simulink model "model"  (R2014a)
(part 3 of 3)

  powergui : powerlib/powergui  Priority=1  SimulationMode=Continuous  SolverType=Tustin  SampleTime=50e-6  frequency=60  SPID=off  DisableSnubberDevices=off  DisableRonSwitches=off  DisableVfSwitches=off  SwTol=0  Interpol=off  DisplayEquations=off  Ts=0  methode=off  frequencyindice=60  Pbase=100e6  ErrMax=1e-4  Iterations=50  UnitsV=kV  UnitsW=MW  FunctionMessages=off  echomessages=off  HookPort=off  EnableUseOfTLC=off  x0status=blocks  RestoreLinks=warning  ResistiveCurrentMeasurement=off  Frange=[0:2:500]  Ylog=off  Xlog=on  ShowGrid=off  save=off  variable=ZData  structure=0  ZoomFFT=off  StartTime=0.0  cycles=1  DisplayStyle=1  fundamental=60  FreqAxis=off  MaxFrequency=1000  frequencyindicesteady=1  RmsSteady=1  display=off
  ВЛ_110_кВ_ВТГРЭС___ПС_Рудянка_CN_276394749_110000_CN_188857424_110000 : powerlib/Elements/Distributed Parameters Line  Phases=3  Frequency=60  Resistance=[0.01273 0.3864]  Inductance="[0.9337e-3  4.1264e-3]"  Capacitance=[12.74e-9 7.751e-9]  Length=27.2985  x1=[0 0 0 0; 0.0001244 0 0 0; 0.0002488 0 0 0; 0.0003733 0 0 0; 0.0004977 0 0 0; 0.0006221 0 0 0]  x2=[0 0 0 0; 0.0001244 0 0 0; 0.0002488 0 0 0; 0.0003733 0 0 0; 0.0004977 0 0 0; 0.0006221 0 0 0]  x3=[0 0 0 0; 0.0001244 0 0 0; 0.0002488 0 0 0; 0.0003733 0 0 0; 0.0004977 0 0 0; 0.0006221 0 0 0]  x4=[0 0 0 0; 0.0001244 0 0 0; 0.0002488 0 0 0; 0.0003733 0 0 0; 0.0004977 0 0 0; 0.0006221 0 0 0]  x5=0  V1=ones(3,3)  V2=ones(3,3)  I1=ones(3,3)  I2=ones(3,3)  nHarmo=1  Measurements=None
  ВЛ_110_кВ_Верховино_Успенка_CN_174028758_110000_CN_277716444_110000 : powerlib/Elements/Distributed Parameters Line  Phases=3  Frequency=60  Resistance=[0.01273 0.3864]  Inductance="[0.9337e-3  4.1264e-3]"  Capacitance=[12.74e-9 7.751e-9]  Length=31.6484  x1=[0 0 0 0; 0.0001244 0 0 0; 0.0002488 0 0 0; 0.0003733 0 0 0; 0.0004977 0 0 0; 0.0006221 0 0 0]  x2=[0 0 0 0; 0.0001244 0 0 0; 0.0002488 0 0 0; 0.0003733 0 0 0; 0.0004977 0 0 0; 0.0006221 0 0 0]  x3=[0 0 0 0; 0.0001244 0 0 0; 0.0002488 0 0 0; 0.0003733 0 0 0; 0.0004977 0 0 0; 0.0006221 0 0 0]  x4=[0 0 0 0; 0.0001244 0 0 0; 0.0002488 0 0 0; 0.0003733 0 0 0; 0.0004977 0 0 0; 0.0006221 0 0 0]  x5=0  V1=ones(3,3)  V2=ones(3,3)  I1=ones(3,3)  I2=ones(3,3)  nHarmo=1  Measurements=None
  ВЛ_110_кВ_Новогеоргиевская___Княженская_CN_373906159_110000_CN_144699678_110000 : powerlib/Elements/Distributed Parameters Line  Phases=3  Frequency=60  Resistance=[0.01273 0.3864]  Inductance="[0.9337e-3  4.1264e-3]"  Capacitance=[12.74e-9 7.751e-9]  Length=16.9419  x1=[0 0 0 0; 0.0001244 0 0 0; 0.0002488 0 0 0; 0.0003733 0 0 0; 0.0004977 0 0 0; 0.0006221 0 0 0]  x2=[0 0 0 0; 0.0001244 0 0 0; 0.0002488 0 0 0; 0.0003733 0 0 0; 0.0004977 0 0 0; 0.0006221 0 0 0]  x3=[0 0 0 0; 0.0001244 0 0 0; 0.0002488 0 0 0; 0.0003733 0 0 0; 0.0004977 0 0 0; 0.0006221 0 0 0]  x4=[0 0 0 0; 0.0001244 0 0 0; 0.0002488 0 0 0; 0.0003733 0 0 0; 0.0004977 0 0 0; 0.0006221 0 0 0]  x5=0  V1=ones(3,3)  V2=ones(3,3)  I1=ones(3,3)  I2=ones(3,3)  nHarmo=1  Measurements=None
  ВЛ_110_кВ_Окунево___Солнечная_1_CN_273707087_110000_CN_110538007_110000 : powerlib/Elements/Distributed Parameters Line  Phases=3  Frequency=60  Resistance=[0.01273 0.3864]  Inductance="[0.9337e-3  4.1264e-3]"  Capacitance=[12.74e-9 7.751e-9]  Length=7.7084  x1=[0 0 0 0; 0.0001244 0 0 0; 0.0002488 0 0 0; 0.0003733 0 0 0; 0.0004977 0 0 0; 0.0006221 0 0 0]  x2=[0 0 0 0; 0.0001244 0 0 0; 0.0002488 0 0 0; 0.0003733 0 0 0; 0.0004977 0 0 0; 0.0006221 0 0 0]  x3=[0 0 0 0; 0.0001244 0 0 0; 0.0002488 0 0 0; 0.0003733 0 0 0; 0.0004977 0 0 0; 0.0006221 0 0 0]  x4=[0 0 0 0; 0.0001244 0 0 0; 0.0002488 0 0 0; 0.0003733 0 0 0; 0.0004977 0 0 0; 0.0006221 0 0 0]  x5=0  V1=ones(3,3)  V2=ones(3,3)  I1=ones(3,3)  I2=ones(3,3)  nHarmo=1  Measurements=None
  ВЛ_110_кВ_ПС_Зарница___ПС_Тугулым_CN_229397794_110000_CN_279664558_110000 : powerlib/Elements/Distributed Parameters Line  Phases=3  Frequency=60  Resistance=[0.01273 0.3864]  Inductance="[0.9337e-3  4.1264e-3]"  Capacitance=[12.74e-9 7.751e-9]  Length=22.5038  x1=[0 0 0 0; 0.0001244 0 0 0; 0.0002488 0 0 0; 0.0003733 0 0 0; 0.0004977 0 0 0; 0.0006221 0 0 0]  x2=[0 0 0 0; 0.0001244 0 0 0; 0.0002488 0 0 0; 0.0003733 0 0 0; 0.0004977 0 0 0; 0.0006221 0 0 0]  x3=[0 0 0 0; 0.0001244 0 0 0; 0.0002488 0 0 0; 0.0003733 0 0 0; 0.0004977 0 0 0; 0.0006221 0 0 0]  x4=[0 0 0 0; 0.0001244 0 0 0; 0.0002488 0 0 0; 0.0003733 0 0 0; 0.0004977 0 0 0; 0.0006221 0 0 0]  x5=0  V1=ones(3,3)  V2=ones(3,3)  I1=ones(3,3)  I2=ones(3,3)  nHarmo=1  Measurements=None
  ВЛ_110_кВ_ПС_Кармак___ПС_Верховино_CN_279664559_110000_CN_174028758_110000 : powerlib/Elements/Distributed Parameters Line  Phases=3  Frequency=60  Resistance=[0.01273 0.3864]  Inductance="[0.9337e-3  4.1264e-3]"  Capacitance=[12.74e-9 7.751e-9]  Length=5.7456  x1=[0 0 0 0; 0.0001244 0 0 0; 0.0002488 0 0 0; 0.0003733 0 0 0; 0.0004977 0 0 0; 0.0006221 0 0 0]  x2=[0 0 0 0; 0.0001244 0 0 0; 0.0002488 0 0 0; 0.0003733 0 0 0; 0.0004977 0 0 0; 0.0006221 0 0 0]  x3=[0 0 0 0; 0.0001244 0 0 0; 0.0002488 0 0 0; 0.0003733 0 0 0; 0.0004977 0 0 0; 0.0006221 0 0 0]  x4=[0 0 0 0; 0.0001244 0 0 0; 0.0002488 0 0 0; 0.0003733 0 0 0; 0.0004977 0 0 0; 0.0006221 0 0 0]  x5=0  V1=ones(3,3)  V2=ones(3,3)  I1=ones(3,3)  I2=ones(3,3)  nHarmo=1  Measurements=None
  ВЛ_110_кВ_ПС_Краснотурьинск___ПС_Североуральск_CN_281458614_110000_CN_281458615_110000 : powerlib/Elements/Distributed Parameters Line  Phases=3  Frequency=60  Resistance=[0.01273 0.3864]  Inductance="[0.9337e-3  4.1264e-3]"  Capacitance=[12.74e-9 7.751e-9]  Length=3.8522  x1=[0 0 0 0; 0.0001244 0 0 0; 0.0002488 0 0 0; 0.0003733 0 0 0; 0.0004977 0 0 0; 0.0006221 0 0 0]  x2=[0 0 0 0; 0.0001244 0 0 0; 0.0002488 0 0 0; 0.0003733 0 0 0; 0.0004977 0 0 0; 0.0006221 0 0 0]  x3=[0 0 0 0; 0.0001244 0 0 0; 0.0002488 0 0 0; 0.0003733 0 0 0; 0.0004977 0 0 0; 0.0006221 0 0 0]  x4=[0 0 0 0; 0.0001244 0 0 0; 0.0002488 0 0 0; 0.0003733 0 0 0; 0.0004977 0 0 0; 0.0006221 0 0 0]  x5=0  V1=ones(3,3)  V2=ones(3,3)  I1=ones(3,3)  I2=ones(3,3)  nHarmo=1  Measurements=None
  ВЛ_110_кВ_ПС_Черемухово___ПС_Першино_CN_235846243_110000_CN_281707739_110000 : powerlib/Elements/Distributed Parameters Line  Phases=3  Frequency=60  Resistance=[0.01273 0.3864]  Inductance="[0.9337e-3  4.1264e-3]"  Capacitance=[12.74e-9 7.751e-9]  Length=9.1519  x1=[0 0 0 0; 0.0001244 0 0 0; 0.0002488 0 0 0; 0.0003733 0 0 0; 0.0004977 0 0 0; 0.0006221 0 0 0]  x2=[0 0 0 0; 0.0001244 0 0 0; 0.0002488 0 0 0; 0.0003733 0 0 0; 0.0004977 0 0 0; 0.0006221 0 0 0]  x3=[0 0 0 0; 0.0001244 0 0 0; 0.0002488 0 0 0; 0.0003733 0 0 0; 0.0004977 0 0 0; 0.0006221 0 0 0]  x4=[0 0 0 0; 0.0001244 0 0 0; 0.0002488 0 0 0; 0.0003733 0 0 0; 0.0004977 0 0 0; 0.0006221 0 0 0]  x5=0  V1=ones(3,3)  V2=ones(3,3)  I1=ones(3,3)  I2=ones(3,3)  nHarmo=1  Measurements=None
  ВЛ_110_кВ_ПС_Черноисточинск___ПС_НЦЗ_CN_105584274_110000_CN_274851642_110000 : powerlib/Elements/Distributed Parameters Line  Phases=3  Frequency=60  Resistance=[0.01273 0.3864]  Inductance="[0.9337e-3  4.1264e-3]"  Capacitance=[12.74e-9 7.751e-9]  Length=49.7933  x1=[0 0 0 0; 0.0001244 0 0 0; 0.0002488 0 0 0; 0.0003733 0 0 0; 0.0004977 0 0 0; 0.0006221 0 0 0]  x2=[0 0 0 0; 0.0001244 0 0 0; 0.0002488 0 0 0; 0.0003733 0 0 0; 0.0004977 0 0 0; 0.0006221 0 0 0]  x3=[0 0 0 0; 0.0001244 0 0 0; 0.0002488 0 0 0; 0.0003733 0 0 0; 0.0004977 0 0 0; 0.0006221 0 0 0]  x4=[0 0 0 0; 0.0001244 0 0 0; 0.0002488 0 0 0; 0.0003733 0 0 0; 0.0004977 0 0 0; 0.0006221 0 0 0]  x5=0  V1=ones(3,3)  V2=ones(3,3)  I1=ones(3,3)  I2=ones(3,3)  nHarmo=1  Measurements=None
  ВЛ_110_кВ_ПС_Школьная___ПС_Рудянка_CN_275095838_110000_CN_276394749_110000 : powerlib/Elements/Distributed Parameters Line  Phases=3  Frequency=60  Resistance=[0.01273 0.3864]  Inductance="[0.9337e-3  4.1264e-3]"  Capacitance=[12.74e-9 7.751e-9]  Length=22.0688  x1=[0 0 0 0; 0.0001244 0 0 0; 0.0002488 0 0 0; 0.0003733 0 0 0; 0.0004977 0 0 0; 0.0006221 0 0 0]  x2=[0 0 0 0; 0.0001244 0 0 0; 0.0002488 0 0 0; 0.0003733 0 0 0; 0.0004977 0 0 0; 0.0006221 0 0 0]  x3=[0 0 0 0; 0.0001244 0 0 0; 0.0002488 0 0 0; 0.0003733 0 0 0; 0.0004977 0 0 0; 0.0006221 0 0 0]  x4=[0 0 0 0; 0.0001244 0 0 0; 0.0002488 0 0 0; 0.0003733 0 0 0; 0.0004977 0 0 0; 0.0006221 0 0 0]  x5=0  V1=ones(3,3)  V2=ones(3,3)  I1=ones(3,3)  I2=ones(3,3)  nHarmo=1  Measurements=None
  ВЛ_110_кВ_ПС_Юшала___ПС_Яр_CN_200241256_110000_CN_279664560_110000 : powerlib/Elements/Distributed Parameters Line  Phases=3  Frequency=60  Resistance=[0.01273 0.3864]  Inductance="[0.9337e-3  4.1264e-3]"  Capacitance=[12.74e-9 7.751e-9]  Length=16.032  x1=[0 0 0 0; 0.0001244 0 0 0; 0.0002488 0 0 0; 0.0003733 0 0 0; 0.0004977 0 0 0; 0.0006221 0 0 0]  x2=[0 0 0 0; 0.0001244 0 0 0; 0.0002488 0 0 0; 0.0003733 0 0 0; 0.0004977 0 0 0; 0.0006221 0 0 0]  x3=[0 0 0 0; 0.0001244 0 0 0; 0.0002488 0 0 0; 0.0003733 0 0 0; 0.0004977 0 0 0; 0.0006221 0 0 0]  x4=[0 0 0 0; 0.0001244 0 0 0; 0.0002488 0 0 0; 0.0003733 0 0 0; 0.0004977 0 0 0; 0.0006221 0 0 0]  x5=0  V1=ones(3,3)  V2=ones(3,3)  I1=ones(3,3)  I2=ones(3,3)  nHarmo=1  Measurements=None
  ВЛ_110_кВ_ПС_Яр___ПС_Истоур_CN_200241256_110000_CN_280145603_110000 : powerlib/Elements/Distributed Parameters Line  Phases=3  Frequency=60  Resistance=[0.01273 0.3864]  Inductance="[0.9337e-3  4.1264e-3]"  Capacitance=[12.74e-9 7.751e-9]  Length=35.0943  x1=[0 0 0 0; 0.0001244 0 0 0; 0.0002488 0 0 0; 0.0003733 0 0 0; 0.0004977 0 0 0; 0.0006221 0 0 0]  x2=[0 0 0 0; 0.0001244 0 0 0; 0.0002488 0 0 0; 0.0003733 0 0 0; 0.0004977 0 0 0; 0.0006221 0 0 0]  x3=[0 0 0 0; 0.0001244 0 0 0; 0.0002488 0 0 0; 0.0003733 0 0 0; 0.0004977 0 0 0; 0.0006221 0 0 0]  x4=[0 0 0 0; 0.0001244 0 0 0; 0.0002488 0 0 0; 0.0003733 0 0 0; 0.0004977 0 0 0; 0.0006221 0 0 0]  x5=0  V1=ones(3,3)  V2=ones(3,3)  I1=ones(3,3)  I2=ones(3,3)  nHarmo=1  Measurements=None
  ВЛ_110_кВ_СУГРЭС___ПС_Школьная_CN_275095838_110000_CN_131114928_110000 : powerlib/Elements/Distributed Parameters Line  Phases=3  Frequency=60  Resistance=[0.01273 0.3864]  Inductance="[0.9337e-3  4.1264e-3]"  Capacitance=[12.74e-9 7.751e-9]  Length=53.717  x1=[0 0 0 0; 0.0001244 0 0 0; 0.0002488 0 0 0; 0.0003733 0 0 0; 0.0004977 0 0 0; 0.0006221 0 0 0]  x2=[0 0 0 0; 0.0001244 0 0 0; 0.0002488 0 0 0; 0.0003733 0 0 0; 0.0004977 0 0 0; 0.0006221 0 0 0]  x3=[0 0 0 0; 0.0001244 0 0 0; 0.0002488 0 0 0; 0.0003733 0 0 0; 0.0004977 0 0 0; 0.0006221 0 0 0]  x4=[0 0 0 0; 0.0001244 0 0 0; 0.0002488 0 0 0; 0.0003733 0 0 0; 0.0004977 0 0 0; 0.0006221 0 0 0]  x5=0  V1=ones(3,3)  V2=ones(3,3)  I1=ones(3,3)  I2=ones(3,3)  nHarmo=1  Measurements=None
  ВЛ_110_кВ_СУГРЭС___ПС_Школьная_CN_275095838_110000_CN_317157140_110000 : powerlib/Elements/Distributed Parameters Line  Phases=3  Frequency=60  Resistance=[0.01273 0.3864]  Inductance="[0.9337e-3  4.1264e-3]"  Capacitance=[12.74e-9 7.751e-9]  Length=32.9199  x1=[0 0 0 0; 0.0001244 0 0 0; 0.0002488 0 0 0; 0.0003733 0 0 0; 0.0004977 0 0 0; 0.0006221 0 0 0]  x2=[0 0 0 0; 0.0001244 0 0 0; 0.0002488 0 0 0; 0.0003733 0 0 0; 0.0004977 0 0 0; 0.0006221 0 0 0]  x3=[0 0 0 0; 0.0001244 0 0 0; 0.0002488 0 0 0; 0.0003733 0 0 0; 0.0004977 0 0 0; 0.0006221 0 0 0]  x4=[0 0 0 0; 0.0001244 0 0 0; 0.0002488 0 0 0; 0.0003733 0 0 0; 0.0004977 0 0 0; 0.0006221 0 0 0]  x5=0  V1=ones(3,3)  V2=ones(3,3)  I1=ones(3,3)  I2=ones(3,3)  nHarmo=1  Measurements=None
  ВЛ_110_кВ_СУГРЭС___ПС_Школьная_CN_275095838_110000_CN_37479179_110000 : powerlib/Elements/Distributed Parameters Line  Phases=3  Frequency=60  Resistance=[0.01273 0.3864]  Inductance="[0.9337e-3  4.1264e-3]"  Capacitance=[12.74e-9 7.751e-9]  Length=30.521  x1=[0 0 0 0; 0.0001244 0 0 0; 0.0002488 0 0 0; 0.0003733 0 0 0; 0.0004977 0 0 0; 0.0006221 0 0 0]  x2=[0 0 0 0; 0.0001244 0 0 0; 0.0002488 0 0 0; 0.0003733 0 0 0; 0.0004977 0 0 0; 0.0006221 0 0 0]  x3=[0 0 0 0; 0.0001244 0 0 0; 0.0002488 0 0 0; 0.0003733 0 0 0; 0.0004977 0 0 0; 0.0006221 0 0 0]  x4=[0 0 0 0; 0.0001244 0 0 0; 0.0002488 0 0 0; 0.0003733 0 0 0; 0.0004977 0 0 0; 0.0006221 0 0 0]  x5=0  V1=ones(3,3)  V2=ones(3,3)  I1=ones(3,3)  I2=ones(3,3)  nHarmo=1  Measurements=None
  ВЛ_110_кВ_СУГРЭС___ПС_Школьная_CN_275095838_110000_CN_66264428_110000 : powerlib/Elements/Distributed Parameters Line  Phases=3  Frequency=60  Resistance=[0.01273 0.3864]  Inductance="[0.9337e-3  4.1264e-3]"  Capacitance=[12.74e-9 7.751e-9]  Length=36.1648  x1=[0 0 0 0; 0.0001244 0 0 0; 0.0002488 0 0 0; 0.0003733 0 0 0; 0.0004977 0 0 0; 0.0006221 0 0 0]  x2=[0 0 0 0; 0.0001244 0 0 0; 0.0002488 0 0 0; 0.0003733 0 0 0; 0.0004977 0 0 0; 0.0006221 0 0 0]  x3=[0 0 0 0; 0.0001244 0 0 0; 0.0002488 0 0 0; 0.0003733 0 0 0; 0.0004977 0 0 0; 0.0006221 0 0 0]  x4=[0 0 0 0; 0.0001244 0 0 0; 0.0002488 0 0 0; 0.0003733 0 0 0; 0.0004977 0 0 0; 0.0006221 0 0 0]  x5=0  V1=ones(3,3)  V2=ones(3,3)  I1=ones(3,3)  I2=ones(3,3)  nHarmo=1  Measurements=None
  ВЛ_110_кВ_СУГРЭС___ПС_Школьная_CN_275095838_110000_CN_76449471_110000 : powerlib/Elements/Distributed Parameters Line  Phases=3  Frequency=60  Resistance=[0.01273 0.3864]  Inductance="[0.9337e-3  4.1264e-3]"  Capacitance=[12.74e-9 7.751e-9]  Length=48.8137  x1=[0 0 0 0; 0.0001244 0 0 0; 0.0002488 0 0 0; 0.0003733 0 0 0; 0.0004977 0 0 0; 0.0006221 0 0 0]  x2=[0 0 0 0; 0.0001244 0 0 0; 0.0002488 0 0 0; 0.0003733 0 0 0; 0.0004977 0 0 0; 0.0006221 0 0 0]  x3=[0 0 0 0; 0.0001244 0 0 0; 0.0002488 0 0 0; 0.0003733 0 0 0; 0.0004977 0 0 0; 0.0006221 0 0 0]  x4=[0 0 0 0; 0.0001244 0 0 0; 0.0002488 0 0 0; 0.0003733 0 0 0; 0.0004977 0 0 0; 0.0006221 0 0 0]  x5=0  V1=ones(3,3)  V2=ones(3,3)  I1=ones(3,3)  I2=ones(3,3)  nHarmo=1  Measurements=None
  ВЛ_110кВ_Кр_Горка_Арси_CN_250194000_110000_CN_191446930_110000 : powerlib/Elements/Distributed Parameters Line  Phases=3  Frequency=60  Resistance=[0.01273 0.3864]  Inductance="[0.9337e-3  4.1264e-3]"  Capacitance=[12.74e-9 7.751e-9]  Length=30.043  x1=[0 0 0 0; 0.0001244 0 0 0; 0.0002488 0 0 0; 0.0003733 0 0 0; 0.0004977 0 0 0; 0.0006221 0 0 0]  x2=[0 0 0 0; 0.0001244 0 0 0; 0.0002488 0 0 0; 0.0003733 0 0 0; 0.0004977 0 0 0; 0.0006221 0 0 0]  x3=[0 0 0 0; 0.0001244 0 0 0; 0.0002488 0 0 0; 0.0003733 0 0 0; 0.0004977 0 0 0; 0.0006221 0 0 0]  x4=[0 0 0 0; 0.0001244 0 0 0; 0.0002488 0 0 0; 0.0003733 0 0 0; 0.0004977 0 0 0; 0.0006221 0 0 0]  x5=0  V1=ones(3,3)  V2=ones(3,3)  I1=ones(3,3)  I2=ones(3,3)  nHarmo=1  Measurements=None
  ВЛ_110кВ_Кр_Горка_Березинская_CN_314008364_110000_CN_191446930_110000 : powerlib/Elements/Distributed Parameters Line  Phases=3  Frequency=60  Resistance=[0.01273 0.3864]  Inductance="[0.9337e-3  4.1264e-3]"  Capacitance=[12.74e-9 7.751e-9]  Length=23.6796  x1=[0 0 0 0; 0.0001244 0 0 0; 0.0002488 0 0 0; 0.0003733 0 0 0; 0.0004977 0 0 0; 0.0006221 0 0 0]  x2=[0 0 0 0; 0.0001244 0 0 0; 0.0002488 0 0 0; 0.0003733 0 0 0; 0.0004977 0 0 0; 0.0006221 0 0 0]  x3=[0 0 0 0; 0.0001244 0 0 0; 0.0002488 0 0 0; 0.0003733 0 0 0; 0.0004977 0 0 0; 0.0006221 0 0 0]  x4=[0 0 0 0; 0.0001244 0 0 0; 0.0002488 0 0 0; 0.0003733 0 0 0; 0.0004977 0 0 0; 0.0006221 0 0 0]  x5=0  V1=ones(3,3)  V2=ones(3,3)  I1=ones(3,3)  I2=ones(3,3)  nHarmo=1  Measurements=None
  ВЛ_110кВ_ПС90_Кр_Горка_отпайка_на_Фершампенуаз_CN_199389117_110000_CN_191446930_110000 : powerlib/Elements/Distributed Parameters Line  Phases=3  Frequency=60  Resistance=[0.01273 0.3864]  Inductance="[0.9337e-3  4.1264e-3]"  Capacitance=[12.74e-9 7.751e-9]  Length=19.2536  x1=[0 0 0 0; 0.0001244 0 0 0; 0.0002488 0 0 0; 0.0003733 0 0 0; 0.0004977 0 0 0; 0.0006221 0 0 0]  x2=[0 0 0 0; 0.0001244 0 0 0; 0.0002488 0 0 0; 0.0003733 0 0 0; 0.0004977 0 0 0; 0.0006221 0 0 0]  x3=[0 0 0 0; 0.0001244 0 0 0; 0.0002488 0 0 0; 0.0003733 0 0 0; 0.0004977 0 0 0; 0.0006221 0 0 0]  x4=[0 0 0 0; 0.0001244 0 0 0; 0.0002488 0 0 0; 0.0003733 0 0 0; 0.0004977 0 0 0; 0.0006221 0 0 0]  x5=0  V1=ones(3,3)  V2=ones(3,3)  I1=ones(3,3)  I2=ones(3,3)  nHarmo=1  Measurements=None
  ВЛ_110кВ_ПС90_Кр_Горка_отпайка_на_Фершампенуаз_CN_199389117_110000_CN_339193644_110000 : powerlib/Elements/Distributed Parameters Line  Phases=3  Frequency=60  Resistance=[0.01273 0.3864]  Inductance="[0.9337e-3  4.1264e-3]"  Capacitance=[12.74e-9 7.751e-9]  Length=37.4111  x1=[0 0 0 0; 0.0001244 0 0 0; 0.0002488 0 0 0; 0.0003733 0 0 0; 0.0004977 0 0 0; 0.0006221 0 0 0]  x2=[0 0 0 0; 0.0001244 0 0 0; 0.0002488 0 0 0; 0.0003733 0 0 0; 0.0004977 0 0 0; 0.0006221 0 0 0]  x3=[0 0 0 0; 0.0001244 0 0 0; 0.0002488 0 0 0; 0.0003733 0 0 0; 0.0004977 0 0 0; 0.0006221 0 0 0]  x4=[0 0 0 0; 0.0001244 0 0 0; 0.0002488 0 0 0; 0.0003733 0 0 0; 0.0004977 0 0 0; 0.0006221 0 0 0]  x5=0  V1=ones(3,3)  V2=ones(3,3)  I1=ones(3,3)  I2=ones(3,3)  nHarmo=1  Measurements=None
  ВЛ_220_кВ_ПС_БАЗ___ПС_Белка_CN_300566433_220000_CN_108718929_220000 : powerlib/Elements/Distributed Parameters Line  Phases=3  Frequency=60  Resistance=[0.01273 0.3864]  Inductance="[0.9337e-3  4.1264e-3]"  Capacitance=[12.74e-9 7.751e-9]  Length=8.0242  x1=[0 0 0 0; 0.0001244 0 0 0; 0.0002488 0 0 0; 0.0003733 0 0 0; 0.0004977 0 0 0; 0.0006221 0 0 0]  x2=[0 0 0 0; 0.0001244 0 0 0; 0.0002488 0 0 0; 0.0003733 0 0 0; 0.0004977 0 0 0; 0.0006221 0 0 0]  x3=[0 0 0 0; 0.0001244 0 0 0; 0.0002488 0 0 0; 0.0003733 0 0 0; 0.0004977 0 0 0; 0.0006221 0 0 0]  x4=[0 0 0 0; 0.0001244 0 0 0; 0.0002488 0 0 0; 0.0003733 0 0 0; 0.0004977 0 0 0; 0.0006221 0 0 0]  x5=0  V1=ones(3,3)  V2=ones(3,3)  I1=ones(3,3)  I2=ones(3,3)  nHarmo=1  Measurements=None
  ВЛ_220_кВ_Первомайская_–_Салда_CN_274851651_220000_CN_107585072_220000 : powerlib/Elements/Distributed Parameters Line  Phases=3  Frequency=60  Resistance=[0.01273 0.3864]  Inductance="[0.9337e-3  4.1264e-3]"  Capacitance=[12.74e-9 7.751e-9]  Length=62.8508  x1=[0 0 0 0; 0.0001244 0 0 0; 0.0002488 0 0 0; 0.0003733 0 0 0; 0.0004977 0 0 0; 0.0006221 0 0 0]  x2=[0 0 0 0; 0.0001244 0 0 0; 0.0002488 0 0 0; 0.0003733 0 0 0; 0.0004977 0 0 0; 0.0006221 0 0 0]  x3=[0 0 0 0; 0.0001244 0 0 0; 0.0002488 0 0 0; 0.0003733 0 0 0; 0.0004977 0 0 0; 0.0006221 0 0 0]  x4=[0 0 0 0; 0.0001244 0 0 0; 0.0002488 0 0 0; 0.0003733 0 0 0; 0.0004977 0 0 0; 0.0006221 0 0 0]  x5=0  V1=ones(3,3)  V2=ones(3,3)  I1=ones(3,3)  I2=ones(3,3)  nHarmo=1  Measurements=None
  ВЛ_220_кВ_Троицкая_ГРЭС___Карталы_CN_96842811_220000_CN_109226934_220000 : powerlib/Elements/Distributed Parameters Line  Phases=3  Frequency=60  Resistance=[0.01273 0.3864]  Inductance="[0.9337e-3  4.1264e-3]"  Capacitance=[12.74e-9 7.751e-9]  Length=59.0733  x1=[0 0 0 0; 0.0001244 0 0 0; 0.0002488 0 0 0; 0.0003733 0 0 0; 0.0004977 0 0 0; 0.0006221 0 0 0]  x2=[0 0 0 0; 0.0001244 0 0 0; 0.0002488 0 0 0; 0.0003733 0 0 0; 0.0004977 0 0 0; 0.0006221 0 0 0]  x3=[0 0 0 0; 0.0001244 0 0 0; 0.0002488 0 0 0; 0.0003733 0 0 0; 0.0004977 0 0 0; 0.0006221 0 0 0]  x4=[0 0 0 0; 0.0001244 0 0 0; 0.0002488 0 0 0; 0.0003733 0 0 0; 0.0004977 0 0 0; 0.0006221 0 0 0]  x5=0  V1=ones(3,3)  V2=ones(3,3)  I1=ones(3,3)  I2=ones(3,3)  nHarmo=1  Measurements=None
  ВЛ_220кВ_Тр_ГРЭС_ПС90_1Л_CN_219112642_220000_CN_109226934_220000 : powerlib/Elements/Distributed Parameters Line  Phases=3  Frequency=60  Resistance=[0.01273 0.3864]  Inductance="[0.9337e-3  4.1264e-3]"  Capacitance=[12.74e-9 7.751e-9]  Length=57.6287  x1=[0 0 0 0; 0.0001244 0 0 0; 0.0002488 0 0 0; 0.0003733 0 0 0; 0.0004977 0 0 0; 0.0006221 0 0 0]  x2=[0 0 0 0; 0.0001244 0 0 0; 0.0002488 0 0 0; 0.0003733 0 0 0; 0.0004977 0 0 0; 0.0006221 0 0 0]  x3=[0 0 0 0; 0.0001244 0 0 0; 0.0002488 0 0 0; 0.0003733 0 0 0; 0.0004977 0 0 0; 0.0006221 0 0 0]  x4=[0 0 0 0; 0.0001244 0 0 0; 0.0002488 0 0 0; 0.0003733 0 0 0; 0.0004977 0 0 0; 0.0006221 0 0 0]  x5=0  V1=ones(3,3)  V2=ones(3,3)  I1=ones(3,3)  I2=ones(3,3)  nHarmo=1  Measurements=None
  ВЛ_500кВ_Кропачево___Приваловская_CN_169556579_500000_CN_113767652_500000 : powerlib/Elements/Distributed Parameters Line  Phases=3  Frequency=60  Resistance=[0.01273 0.3864]  Inductance="[0.9337e-3  4.1264e-3]"  Capacitance=[12.74e-9 7.751e-9]  Length=57.2159  x1=[0 0 0 0; 0.0001244 0 0 0; 0.0002488 0 0 0; 0.0003733 0 0 0; 0.0004977 0 0 0; 0.0006221 0 0 0]  x2=[0 0 0 0; 0.0001244 0 0 0; 0.0002488 0 0 0; 0.0003733 0 0 0; 0.0004977 0 0 0; 0.0006221 0 0 0]  x3=[0 0 0 0; 0.0001244 0 0 0; 0.0002488 0 0 0; 0.0003733 0 0 0; 0.0004977 0 0 0; 0.0006221 0 0 0]  x4=[0 0 0 0; 0.0001244 0 0 0; 0.0002488 0 0 0; 0.0003733 0 0 0; 0.0004977 0 0 0; 0.0006221 0 0 0]  x5=0  V1=ones(3,3)  V2=ones(3,3)  I1=ones(3,3)  I2=ones(3,3)  nHarmo=1  Measurements=None
  Отпайка_ВЛ_110_кВ_на_ПС_Твёрдые_сплавы_от_ВТГРЭС___Карпушиха_CN_276394758_110000_CN_188857424_110000 : powerlib/Elements/Distributed Parameters Line  Phases=3  Frequency=60  Resistance=[0.01273 0.3864]  Inductance="[0.9337e-3  4.1264e-3]"  Capacitance=[12.74e-9 7.751e-9]  Length=30.2501  x1=[0 0 0 0; 0.0001244 0 0 0; 0.0002488 0 0 0; 0.0003733 0 0 0; 0.0004977 0 0 0; 0.0006221 0 0 0]  x2=[0 0 0 0; 0.0001244 0 0 0; 0.0002488 0 0 0; 0.0003733 0 0 0; 0.0004977 0 0 0; 0.0006221 0 0 0]  x3=[0 0 0 0; 0.0001244 0 0 0; 0.0002488 0 0 0; 0.0003733 0 0 0; 0.0004977 0 0 0; 0.0006221 0 0 0]  x4=[0 0 0 0; 0.0001244 0 0 0; 0.0002488 0 0 0; 0.0003733 0 0 0; 0.0004977 0 0 0; 0.0006221 0 0 0]  x5=0  V1=ones(3,3)  V2=ones(3,3)  I1=ones(3,3)  I2=ones(3,3)  nHarmo=1  Measurements=None
  ПС_Таволги___ПС_Киприно___ПС_Черемисска_CN_273461546_110000_CN_101532642_110000 : powerlib/Elements/Distributed Parameters Line  Phases=3  Frequency=60  Resistance=[0.01273 0.3864]  Inductance="[0.9337e-3  4.1264e-3]"  Capacitance=[12.74e-9 7.751e-9]  Length=22.6465  x1=[0 0 0 0; 0.0001244 0 0 0; 0.0002488 0 0 0; 0.0003733 0 0 0; 0.0004977 0 0 0; 0.0006221 0 0 0]  x2=[0 0 0 0; 0.0001244 0 0 0; 0.0002488 0 0 0; 0.0003733 0 0 0; 0.0004977 0 0 0; 0.0006221 0 0 0]  x3=[0 0 0 0; 0.0001244 0 0 0; 0.0002488 0 0 0; 0.0003733 0 0 0; 0.0004977 0 0 0; 0.0006221 0 0 0]  x4=[0 0 0 0; 0.0001244 0 0 0; 0.0002488 0 0 0; 0.0003733 0 0 0; 0.0004977 0 0 0; 0.0006221 0 0 0]  x5=0  V1=ones(3,3)  V2=ones(3,3)  I1=ones(3,3)  I2=ones(3,3)  nHarmo=1  Measurements=None
  ПС_Таволги___ПС_Киприно___ПС_Черемисска_CN_273461546_110000_CN_135780398_110000 : powerlib/Elements/Distributed Parameters Line  Phases=3  Frequency=60  Resistance=[0.01273 0.3864]  Inductance="[0.9337e-3  4.1264e-3]"  Capacitance=[12.74e-9 7.751e-9]  Length=26.7512  x1=[0 0 0 0; 0.0001244 0 0 0; 0.0002488 0 0 0; 0.0003733 0 0 0; 0.0004977 0 0 0; 0.0006221 0 0 0]  x2=[0 0 0 0; 0.0001244 0 0 0; 0.0002488 0 0 0; 0.0003733 0 0 0; 0.0004977 0 0 0; 0.0006221 0 0 0]  x3=[0 0 0 0; 0.0001244 0 0 0; 0.0002488 0 0 0; 0.0003733 0 0 0; 0.0004977 0 0 0; 0.0006221 0 0 0]  x4=[0 0 0 0; 0.0001244 0 0 0; 0.0002488 0 0 0; 0.0003733 0 0 0; 0.0004977 0 0 0; 0.0006221 0 0 0]  x5=0  V1=ones(3,3)  V2=ones(3,3)  I1=ones(3,3)  I2=ones(3,3)  nHarmo=1  Measurements=None
  ПС_Таволги___ПС_Киприно___ПС_Черемисска_CN_273461546_110000_CN_273649961_110000 : powerlib/Elements/Distributed Parameters Line  Phases=3  Frequency=60  Resistance=[0.01273 0.3864]  Inductance="[0.9337e-3  4.1264e-3]"  Capacitance=[12.74e-9 7.751e-9]  Length=19.5309  x1=[0 0 0 0; 0.0001244 0 0 0; 0.0002488 0 0 0; 0.0003733 0 0 0; 0.0004977 0 0 0; 0.0006221 0 0 0]  x2=[0 0 0 0; 0.0001244 0 0 0; 0.0002488 0 0 0; 0.0003733 0 0 0; 0.0004977 0 0 0; 0.0006221 0 0 0]  x3=[0 0 0 0; 0.0001244 0 0 0; 0.0002488 0 0 0; 0.0003733 0 0 0; 0.0004977 0 0 0; 0.0006221 0 0 0]  x4=[0 0 0 0; 0.0001244 0 0 0; 0.0002488 0 0 0; 0.0003733 0 0 0; 0.0004977 0 0 0; 0.0006221 0 0 0]  x5=0  V1=ones(3,3)  V2=ones(3,3)  I1=ones(3,3)  I2=ones(3,3)  nHarmo=1  Measurements=None
  Тр_ГРЭС_Магнитогорск_CN_219112646_500000_CN_109226934_220000 : powerlib/Elements/Distributed Parameters Line  Phases=3  Frequency=60  Resistance=[0.01273 0.3864]  Inductance="[0.9337e-3  4.1264e-3]"  Capacitance=[12.74e-9 7.751e-9]  Length=9.2123  x1=[0 0 0 0; 0.0001244 0 0 0; 0.0002488 0 0 0; 0.0003733 0 0 0; 0.0004977 0 0 0; 0.0006221 0 0 0]  x2=[0 0 0 0; 0.0001244 0 0 0; 0.0002488 0 0 0; 0.0003733 0 0 0; 0.0004977 0 0 0; 0.0006221 0 0 0]  x3=[0 0 0 0; 0.0001244 0 0 0; 0.0002488 0 0 0; 0.0003733 0 0 0; 0.0004977 0 0 0; 0.0006221 0 0 0]  x4=[0 0 0 0; 0.0001244 0 0 0; 0.0002488 0 0 0; 0.0003733 0 0 0; 0.0004977 0 0 0; 0.0006221 0 0 0]  x5=0  V1=ones(3,3)  V2=ones(3,3)  I1=ones(3,3)  I2=ones(3,3)  nHarmo=1  Measurements=None
  connections:
  _CN_218733056_110000_CN_218733818_110000/LConn1 -- T_218733056__/LConn1 -- _CN_218733056_110000_CN_218733820_110000/LConn1
  _CN_218733056_110000_CN_218733818_110000/LConn2 -- T_218733056__/LConn2 -- _CN_218733056_110000_CN_218733820_110000/LConn2
  _CN_218733056_110000_CN_218733818_110000/LConn3 -- T_218733056__/LConn3 -- _CN_218733056_110000_CN_218733820_110000/LConn3 -- bus1/LConn1
  T_218733818__/LConn1 -- _CN_218733056_110000_CN_218733818_110000/RConn1
  T_218733818__/LConn2 -- _CN_218733056_110000_CN_218733818_110000/RConn2
  _CN_218733056_110000_CN_218733818_110000/RConn3 -- T_218733818__/LConn3 -- bus2/LConn1
  T_218733820__/LConn1 -- _CN_218733056_110000_CN_218733820_110000/RConn1
  T_218733820__/LConn2 -- _CN_218733056_110000_CN_218733820_110000/RConn2
  _CN_218733056_110000_CN_218733820_110000/RConn3 -- T_218733820__/LConn3 -- bus3/LConn1
  _CN_128448427_110000_CN_40080294_110000/LConn1 -- T_128448427__/LConn1 -- _CN_128448427_110000_CN_42918338_110000/LConn1 -- _CN_128448427_110000_CN_310639917_110000/LConn1 -- _CN_128448427_110000_CN_78488044_110000/LConn1 -- _CN_128448427_110000_CN_97827873_110000/LConn1
  _CN_128448427_110000_CN_40080294_110000/LConn2 -- T_128448427__/LConn2 -- _CN_128448427_110000_CN_42918338_110000/LConn2 -- _CN_128448427_110000_CN_310639917_110000/LConn2 -- _CN_128448427_110000_CN_78488044_110000/LConn2 -- _CN_128448427_110000_CN_97827873_110000/LConn2
  _CN_128448427_110000_CN_40080294_110000/LConn3 -- T_128448427__/LConn3 -- _CN_128448427_110000_CN_42918338_110000/LConn3 -- bus4/LConn1 -- _CN_128448427_110000_CN_310639917_110000/LConn3 -- _CN_128448427_110000_CN_78488044_110000/LConn3 -- _CN_128448427_110000_CN_97827873_110000/LConn3
  T_40080294_110000;10000_Московская/LConn1 -- _CN_128448427_110000_CN_40080294_110000/RConn1
  T_40080294_110000;10000_Московская/LConn2 -- _CN_128448427_110000_CN_40080294_110000/RConn2
  _CN_128448427_110000_CN_40080294_110000/RConn3 -- T_40080294_110000;10000_Московская/LConn3 -- bus5/LConn1
  T_310639917_110000;10000_Отрадная/LConn1 -- _CN_128448427_110000_CN_310639917_110000/RConn1
  T_310639917_110000;10000_Отрадная/LConn2 -- _CN_128448427_110000_CN_310639917_110000/RConn2
  _CN_128448427_110000_CN_310639917_110000/RConn3 -- T_310639917_110000;10000_Отрадная/LConn3 -- bus6/LConn1
  T_78488044__Академическая/LConn1 -- _CN_128448427_110000_CN_78488044_110000/RConn1
  T_78488044__Академическая/LConn2 -- _CN_128448427_110000_CN_78488044_110000/RConn2
  _CN_128448427_110000_CN_78488044_110000/RConn3 -- T_78488044__Академическая/LConn3 -- bus7/LConn1
  T_97827873__Овощная/LConn1 -- _CN_128448427_110000_CN_97827873_110000/RConn1
  T_97827873__Овощная/LConn2 -- _CN_128448427_110000_CN_97827873_110000/RConn2
  _CN_128448427_110000_CN_97827873_110000/RConn3 -- T_97827873__Овощная/LConn3 -- bus8/LConn1
  T_42918338__Ясная/LConn1 -- _CN_128448427_110000_CN_42918338_110000/RConn1
  T_42918338__Ясная/LConn2 -- _CN_128448427_110000_CN_42918338_110000/RConn2
  _CN_128448427_110000_CN_42918338_110000/RConn3 -- T_42918338__Ясная/LConn3 -- bus9/LConn1
  _CN_331102892_110000_CN_128346488_110000/LConn1 -- T_331102892__Бараба/LConn1 -- _CN_331102892_110000_CN_164371995_110000/LConn1 -- _CN_331102892_110000_CN_187971431_110000/LConn1 -- _CN_331102892_110000_CN_93050981_110000/LConn1
  _CN_331102892_110000_CN_128346488_110000/LConn2 -- T_331102892__Бараба/LConn2 -- _CN_331102892_110000_CN_164371995_110000/LConn2 -- _CN_331102892_110000_CN_187971431_110000/LConn2 -- _CN_331102892_110000_CN_93050981_110000/LConn2
  _CN_331102892_110000_CN_128346488_110000/LConn3 -- T_331102892__Бараба/LConn3 -- _CN_331102892_110000_CN_164371995_110000/LConn3 -- _CN_331102892_110000_CN_187971431_110000/LConn3 -- _CN_331102892_110000_CN_93050981_110000/LConn3 -- bus10/LConn1
  T_128346488__Грязновская/LConn1 -- _CN_331102892_110000_CN_128346488_110000/RConn1
  T_128346488__Грязновская/LConn2 -- _CN_331102892_110000_CN_128346488_110000/RConn2
  _CN_331102892_110000_CN_128346488_110000/RConn3 -- T_128346488__Грязновская/LConn3 -- bus11/LConn1
  T_164371995__/LConn1 -- _CN_331102892_110000_CN_164371995_110000/RConn1
  T_164371995__/LConn2 -- _CN_331102892_110000_CN_164371995_110000/RConn2
  _CN_331102892_110000_CN_164371995_110000/RConn3 -- T_164371995__/LConn3 -- bus12/LConn1
  T_187971431__Клевакино/LConn1 -- _CN_331102892_110000_CN_187971431_110000/RConn1
  T_187971431__Клевакино/LConn2 -- _CN_331102892_110000_CN_187971431_110000/RConn2
  _CN_331102892_110000_CN_187971431_110000/RConn3 -- T_187971431__Клевакино/LConn3 -- bus13/LConn1
  _CN_331102892_110000_CN_93050981_110000/RConn1 -- T_93050981__Черемхово/LConn1 -- _CN_320347053_110000_CN_93050981_110000/LConn1
  _CN_331102892_110000_CN_93050981_110000/RConn2 -- T_93050981__Черемхово/LConn2 -- _CN_320347053_110000_CN_93050981_110000/LConn2
  _CN_331102892_110000_CN_93050981_110000/RConn3 -- T_93050981__Черемхово/LConn3 -- _CN_320347053_110000_CN_93050981_110000/LConn3 -- bus14/LConn1
  T_320347053__Кочневское/LConn1 -- _CN_320347053_110000_CN_93050981_110000/RConn1
  T_320347053__Кочневское/LConn2 -- _CN_320347053_110000_CN_93050981_110000/RConn2
  _CN_320347053_110000_CN_93050981_110000/RConn3 -- T_320347053__Кочневское/LConn3 -- bus15/LConn1
  T_279497233__/LConn1 -- _CN_279497233_110000_CN_126093674_110000/LConn1
  T_279497233__/LConn2 -- _CN_279497233_110000_CN_126093674_110000/LConn2
  _CN_279497233_110000_CN_126093674_110000/LConn3 -- T_279497233__/LConn3 -- bus16/LConn1
  T_126093674__/LConn1 -- _CN_279497233_110000_CN_126093674_110000/RConn1
  T_126093674__/LConn2 -- _CN_279497233_110000_CN_126093674_110000/RConn2
  _CN_279497233_110000_CN_126093674_110000/RConn3 -- T_126093674__/LConn3 -- bus17/LConn1
  "T_96989715_110000;6000_ПС_\"Кварц\""/LConn1 -- _CN_96989715_110000_CN_93260139_110000/LConn1
  "T_96989715_110000;6000_ПС_\"Кварц\""/LConn2 -- _CN_96989715_110000_CN_93260139_110000/LConn2
  _CN_96989715_110000_CN_93260139_110000/LConn3 -- "T_96989715_110000;6000_ПС_\"Кварц\""/LConn3 -- bus18/LConn1
  T_93260139__Родник/LConn1 -- _CN_96989715_110000_CN_93260139_110000/RConn1
  T_93260139__Родник/LConn2 -- _CN_96989715_110000_CN_93260139_110000/RConn2
  _CN_96989715_110000_CN_93260139_110000/RConn3 -- T_93260139__Родник/LConn3 -- bus19/LConn1
  _CN_274652249_110000_CN_216208030_110000/LConn1 -- "T_274652249__П_ст_110_35_6кВ_\"Атиг\""/LConn1 -- _CN_274652249_110000_CN_106927870_110000/LConn1 -- _CN_274652249_110000_CN_255624915_110000/LConn1
  _CN_274652249_110000_CN_216208030_110000/LConn2 -- "T_274652249__П_ст_110_35_6кВ_\"Атиг\""/LConn2 -- _CN_274652249_110000_CN_106927870_110000/LConn2 -- _CN_274652249_110000_CN_255624915_110000/LConn2
  _CN_274652249_110000_CN_216208030_110000/LConn3 -- "T_274652249__П_ст_110_35_6кВ_\"Атиг\""/LConn3 -- _CN_274652249_110000_CN_106927870_110000/LConn3 -- _CN_274652249_110000_CN_255624915_110000/LConn3 -- bus20/LConn1
  "T_216208030_110000;35000;6000_ПС_\"Бисерть\""/LConn1 -- _CN_274652249_110000_CN_216208030_110000/RConn1
  "T_216208030_110000;35000;6000_ПС_\"Бисерть\""/LConn2 -- _CN_274652249_110000_CN_216208030_110000/RConn2
  _CN_274652249_110000_CN_216208030_110000/RConn3 -- "T_216208030_110000;35000;6000_ПС_\"Бисерть\""/LConn3 -- bus21/LConn1
  _CN_274652249_110000_CN_106927870_110000/RConn1 -- T_106927870__/LConn1 -- _CN_255624915_110000_CN_106927870_110000/LConn1
  _CN_274652249_110000_CN_106927870_110000/RConn2 -- T_106927870__/LConn2 -- _CN_255624915_110000_CN_106927870_110000/LConn2
  _CN_274652249_110000_CN_106927870_110000/RConn3 -- T_106927870__/LConn3 -- _CN_255624915_110000_CN_106927870_110000/LConn3 -- bus22/LConn1
  _CN_274652249_110000_CN_255624915_110000/RConn1 -- T_255624915__/LConn1 -- _CN_255624915_110000_CN_106927870_110000/RConn1
  _CN_274652249_110000_CN_255624915_110000/RConn2 -- T_255624915__/LConn2 -- _CN_255624915_110000_CN_106927870_110000/RConn2
  _CN_274652249_110000_CN_255624915_110000/RConn3 -- T_255624915__/LConn3 -- _CN_255624915_110000_CN_106927870_110000/RConn3 -- bus23/LConn1
  T_153740317_110000_ГОРНЫЙ_ЩИТ/LConn1 -- _CN_153740317_110000_CN_153741014_110000/LConn1
  T_153740317_110000_ГОРНЫЙ_ЩИТ/LConn2 -- _CN_153740317_110000_CN_153741014_110000/LConn2
  _CN_153740317_110000_CN_153741014_110000/LConn3 -- T_153740317_110000_ГОРНЫЙ_ЩИТ/LConn3 -- bus24/LConn1
  T_153741014__/LConn1 -- _CN_153740317_110000_CN_153741014_110000/RConn1
  T_153741014__/LConn2 -- _CN_153740317_110000_CN_153741014_110000/RConn2
  _CN_153740317_110000_CN_153741014_110000/RConn3 -- T_153741014__/LConn3 -- bus25/LConn1
  _CN_282779585_110000_CN_93418566_110000/LConn1 -- T_282779585__/LConn1 -- _CN_282779585_110000_CN_282779587_110000/LConn1
  _CN_282779585_110000_CN_93418566_110000/LConn2 -- T_282779585__/LConn2 -- _CN_282779585_110000_CN_282779587_110000/LConn2
  _CN_282779585_110000_CN_93418566_110000/LConn3 -- T_282779585__/LConn3 -- _CN_282779585_110000_CN_282779587_110000/LConn3 -- bus26/LConn1
  _CN_282779585_110000_CN_93418566_110000/RConn1 -- T_93418566_220000;110000_Травянская/RConn1 -- _CN_93418566_110000_CN_166188874_110000/LConn1 -- L_93418566/LConn1
  _CN_282779585_110000_CN_93418566_110000/RConn2 -- T_93418566_220000;110000_Травянская/RConn2 -- _CN_93418566_110000_CN_166188874_110000/LConn2 -- L_93418566/LConn2
  _CN_282779585_110000_CN_93418566_110000/RConn3 -- T_93418566_220000;110000_Травянская/RConn3 -- _CN_93418566_110000_CN_166188874_110000/LConn3 -- L_93418566/LConn3 -- bus27/LConn1
  T_282779587__/LConn1 -- _CN_282779585_110000_CN_282779587_110000/RConn1
  T_282779587__/LConn2 -- _CN_282779585_110000_CN_282779587_110000/RConn2
  _CN_282779585_110000_CN_282779587_110000/RConn3 -- T_282779587__/LConn3 -- bus28/LConn1
  T_282645278__/LConn1 -- _CN_282645278_110000_CN_166188874_110000/LConn1
  T_282645278__/LConn2 -- _CN_282645278_110000_CN_166188874_110000/LConn2
  _CN_282645278_110000_CN_166188874_110000/LConn3 -- T_282645278__/LConn3 -- bus29/LConn1
  _CN_282645278_110000_CN_166188874_110000/RConn1 -- T_166188874_220000;110000;10000_Каменская/RConn1 -- _CN_166188874_110000_CN_92045303_110000/LConn1 -- L_166188874/LConn1 -- _CN_166188874_110000_CN_282850239_110000/LConn1 -- _CN_166188874_110000_CN_282748778_110000/LConn1 -- _CN_93418566_110000_CN_166188874_110000/RConn1 -- _CN_280421437_110000_CN_166188874_110000/LConn1
  _CN_282645278_110000_CN_166188874_110000/RConn2 -- T_166188874_220000;110000;10000_Каменская/RConn2 -- _CN_166188874_110000_CN_92045303_110000/LConn2 -- L_166188874/LConn2 -- _CN_166188874_110000_CN_282850239_110000/LConn2 -- _CN_166188874_110000_CN_282748778_110000/LConn2 -- _CN_93418566_110000_CN_166188874_110000/RConn2 -- _CN_280421437_110000_CN_166188874_110000/LConn2
  _CN_282645278_110000_CN_166188874_110000/RConn3 -- T_166188874_220000;110000;10000_Каменская/RConn3 -- _CN_166188874_110000_CN_92045303_110000/LConn3 -- L_166188874/LConn3 -- bus30/LConn1 -- _CN_166188874_110000_CN_282850239_110000/LConn3 -- _CN_166188874_110000_CN_282748778_110000/LConn3 -- _CN_93418566_110000_CN_166188874_110000/RConn3 -- _CN_280421437_110000_CN_166188874_110000/LConn3
  _CN_121211432_110000_CN_372580506_110000/LConn1 -- T_121211432__Ильменская/LConn1 -- _CN_121211432_110000_CN_372580526_110000/LConn1 -- _CN_121211432_110000_CN_116299140_110000/LConn1 -- _CN_121211432_110000_CN_189890975_110000/LConn1
  _CN_121211432_110000_CN_372580506_110000/LConn2 -- T_121211432__Ильменская/LConn2 -- _CN_121211432_110000_CN_372580526_110000/LConn2 -- _CN_121211432_110000_CN_116299140_110000/LConn2 -- _CN_121211432_110000_CN_189890975_110000/LConn2
  _CN_121211432_110000_CN_372580506_110000/LConn3 -- T_121211432__Ильменская/LConn3 -- _CN_121211432_110000_CN_372580526_110000/LConn3 -- _CN_121211432_110000_CN_116299140_110000/LConn3 -- _CN_121211432_110000_CN_189890975_110000/LConn3 -- bus31/LConn1
  _CN_121211432_110000_CN_372580506_110000/RConn1 -- T_372580506_110000_Кулуево/LConn1 -- _CN_372580506_110000_CN_98423617_110000/LConn1
  _CN_121211432_110000_CN_372580506_110000/RConn2 -- T_372580506_110000_Кулуево/LConn2 -- _CN_372580506_110000_CN_98423617_110000/LConn2
  _CN_121211432_110000_CN_372580506_110000/RConn3 -- T_372580506_110000_Кулуево/LConn3 -- _CN_372580506_110000_CN_98423617_110000/LConn3 -- bus32/LConn1
  T_372580526_110000_Яраткулова/LConn1 -- _CN_121211432_110000_CN_372580526_110000/RConn1
  T_372580526_110000_Яраткулова/LConn2 -- _CN_121211432_110000_CN_372580526_110000/RConn2
  _CN_121211432_110000_CN_372580526_110000/RConn3 -- T_372580526_110000_Яраткулова/LConn3 -- bus33/LConn1
  _CN_121211432_110000_CN_116299140_110000/RConn1 -- T_116299140_110000_Чебаркуль/LConn1 -- _CN_361265069_110000_CN_116299140_110000/LConn1 -- _CN_361264295_110000_CN_116299140_110000/LConn1 -- _CN_286951577_110000_CN_116299140_110000/LConn1 -- _CN_361266572_110000_CN_116299140_110000/LConn1
  _CN_121211432_110000_CN_116299140_110000/RConn2 -- T_116299140_110000_Чебаркуль/LConn2 -- _CN_361265069_110000_CN_116299140_110000/LConn2 -- _CN_361264295_110000_CN_116299140_110000/LConn2 -- _CN_286951577_110000_CN_116299140_110000/LConn2 -- _CN_361266572_110000_CN_116299140_110000/LConn2
  _CN_121211432_110000_CN_116299140_110000/RConn3 -- T_116299140_110000_Чебаркуль/LConn3 -- _CN_361265069_110000_CN_116299140_110000/LConn3 -- _CN_361264295_110000_CN_116299140_110000/LConn3 -- bus34/LConn1 -- _CN_286951577_110000_CN_116299140_110000/LConn3 -- _CN_361266572_110000_CN_116299140_110000/LConn3
  _CN_121211432_110000_CN_189890975_110000/RConn1 -- T_189890975_110000_Тургояк/LConn1 -- _CN_144437268_110000_CN_189890975_110000/LConn1 -- _CN_189890975_110000_CN_189890976_110000/LConn1
  _CN_121211432_110000_CN_189890975_110000/RConn2 -- T_189890975_110000_Тургояк/LConn2 -- _CN_144437268_110000_CN_189890975_110000/LConn2 -- _CN_189890975_110000_CN_189890976_110000/LConn2
  _CN_121211432_110000_CN_189890975_110000/RConn3 -- T_189890975_110000_Тургояк/LConn3 -- _CN_144437268_110000_CN_189890975_110000/LConn3 -- _CN_189890975_110000_CN_189890976_110000/LConn3 -- bus35/LConn1
  _CN_115954225_110000_CN_115981920_110000/LConn1 -- "T_115954225__ПС_\"Сухоборка\"_110_10"/LConn1 -- _CN_115954225_110000_CN_115951342_110000/LConn1 -- _CN_115954225_110000_CN_117325674_110000/LConn1
  _CN_115954225_110000_CN_115981920_110000/LConn2 -- "T_115954225__ПС_\"Сухоборка\"_110_10"/LConn2 -- _CN_115954225_110000_CN_115951342_110000/LConn2 -- _CN_115954225_110000_CN_117325674_110000/LConn2
  _CN_115954225_110000_CN_115981920_110000/LConn3 -- "T_115954225__ПС_\"Сухоборка\"_110_10"/LConn3 -- _CN_115954225_110000_CN_115951342_110000/LConn3 -- _CN_115954225_110000_CN_117325674_110000/LConn3 -- bus36/LConn1
  _CN_115954225_110000_CN_115981920_110000/RConn1 -- "T_115981920__ПС_\"Щучье_тяга\"_110_10"/LConn1 -- _CN_115981920_110000_CN_117325672_110000/LConn1 -- _CN_115981920_110000_CN_117325678_110000/LConn1
  _CN_115954225_110000_CN_115981920_110000/RConn2 -- "T_115981920__ПС_\"Щучье_тяга\"_110_10"/LConn2 -- _CN_115981920_110000_CN_117325672_110000/LConn2 -- _CN_115981920_110000_CN_117325678_110000/LConn2
  _CN_115954225_110000_CN_115981920_110000/RConn3 -- "T_115981920__ПС_\"Щучье_тяга\"_110_10"/LConn3 -- _CN_115981920_110000_CN_117325672_110000/LConn3 -- _CN_115981920_110000_CN_117325678_110000/LConn3 -- bus37/LConn1
  "T_115951342__ПС_\"Нифанка\"_110_10"/LConn1 -- _CN_115954225_110000_CN_115951342_110000/RConn1
  "T_115951342__ПС_\"Нифанка\"_110_10"/LConn2 -- _CN_115954225_110000_CN_115951342_110000/RConn2
  _CN_115954225_110000_CN_115951342_110000/RConn3 -- "T_115951342__ПС_\"Нифанка\"_110_10"/LConn3 -- bus38/LConn1
  _CN_115954225_110000_CN_117325674_110000/RConn1 -- "T_117325674__ПС_\"Сафакулево\"_110_10"/LConn1 -- _CN_117325674_110000_CN_117941027_110000/LConn1
  _CN_115954225_110000_CN_117325674_110000/RConn2 -- "T_117325674__ПС_\"Сафакулево\"_110_10"/LConn2 -- _CN_117325674_110000_CN_117941027_110000/LConn2
  _CN_115954225_110000_CN_117325674_110000/RConn3 -- "T_117325674__ПС_\"Сафакулево\"_110_10"/LConn3 -- _CN_117325674_110000_CN_117941027_110000/LConn3 -- bus39/LConn1
  T_144702516__/LConn1 -- _CN_144702516_110000_CN_163401683_110000/LConn1
  T_144702516__/LConn2 -- _CN_144702516_110000_CN_163401683_110000/LConn2
  _CN_144702516_110000_CN_163401683_110000/LConn3 -- T_144702516__/LConn3 -- bus40/LConn1
  _CN_144702516_110000_CN_163401683_110000/RConn1 -- T_163401683_110000_Бреды/LConn1 -- _CN_386978254_110000_CN_163401683_110000/LConn1
  _CN_144702516_110000_CN_163401683_110000/RConn2 -- T_163401683_110000_Бреды/LConn2 -- _CN_386978254_110000_CN_163401683_110000/LConn2
  _CN_144702516_110000_CN_163401683_110000/RConn3 -- T_163401683_110000_Бреды/LConn3 -- _CN_386978254_110000_CN_163401683_110000/LConn3 -- bus41/LConn1
  T_286951577_110000_/LConn1 -- _CN_286951577_110000_CN_116299140_110000/RConn1
  T_286951577_110000_/LConn2 -- _CN_286951577_110000_CN_116299140_110000/RConn2
  _CN_286951577_110000_CN_116299140_110000/RConn3 -- T_286951577_110000_/LConn3 -- bus42/LConn1
  _CN_96842811_110000_CN_254457038_110000/LConn1 -- T_96842811_110000_Карталы/RConn1 -- _CN_96842811_110000_CN_351136526_110000/LConn1 -- L_96842811/LConn1
  _CN_96842811_110000_CN_254457038_110000/LConn2 -- T_96842811_110000_Карталы/RConn2 -- _CN_96842811_110000_CN_351136526_110000/LConn2 -- L_96842811/LConn2
  _CN_96842811_110000_CN_254457038_110000/LConn3 -- T_96842811_110000_Карталы/RConn3 -- _CN_96842811_110000_CN_351136526_110000/LConn3 -- L_96842811/LConn3 -- bus43/LConn1
  T_254457038_110000_Аненская/LConn1 -- _CN_96842811_110000_CN_254457038_110000/RConn1
  T_254457038_110000_Аненская/LConn2 -- _CN_96842811_110000_CN_254457038_110000/RConn2
  _CN_96842811_110000_CN_254457038_110000/RConn3 -- T_254457038_110000_Аненская/LConn3 -- bus44/LConn1
  T_351136526_110000_/LConn1 -- _CN_96842811_110000_CN_351136526_110000/RConn1
  T_351136526_110000_/LConn2 -- _CN_96842811_110000_CN_351136526_110000/RConn2
  _CN_96842811_110000_CN_351136526_110000/RConn3 -- T_351136526_110000_/LConn3 -- bus45/LConn1
  T_280421437__/LConn1 -- _CN_280421437_110000_CN_166188874_110000/RConn1
  T_280421437__/LConn2 -- _CN_280421437_110000_CN_166188874_110000/RConn2
  _CN_280421437_110000_CN_166188874_110000/RConn3 -- T_280421437__/LConn3 -- bus46/LConn1
  ВЛ_110_кВ_СУГРЭС___ПС_Школьная_CN_275095838_110000_CN_37479179_110000/LConn1 -- T_275095838_110000;10000_Школьная/LConn1 -- ВЛ_110_кВ_СУГРЭС___ПС_Школьная_CN_275095838_110000_CN_76449471_110000/LConn1 -- ВЛ_110_кВ_СУГРЭС___ПС_Школьная_CN_275095838_110000_CN_66264428_110000/LConn1 -- ВЛ_110_кВ_СУГРЭС___ПС_Школьная_CN_275095838_110000_CN_131114928_110000/LConn1 -- ВЛ_110_кВ_СУГРЭС___ПС_Школьная_CN_275095838_110000_CN_317157140_110000/LConn1 -- ВЛ_110_кВ_ПС_Школьная___ПС_Рудянка_CN_275095838_110000_CN_276394749_110000/LConn1
  ВЛ_110_кВ_СУГРЭС___ПС_Школьная_CN_275095838_110000_CN_37479179_110000/LConn2 -- T_275095838_110000;10000_Школьная/LConn2 -- ВЛ_110_кВ_СУГРЭС___ПС_Школьная_CN_275095838_110000_CN_76449471_110000/LConn2 -- ВЛ_110_кВ_СУГРЭС___ПС_Школьная_CN_275095838_110000_CN_66264428_110000/LConn2 -- ВЛ_110_кВ_СУГРЭС___ПС_Школьная_CN_275095838_110000_CN_131114928_110000/LConn2 -- ВЛ_110_кВ_СУГРЭС___ПС_Школьная_CN_275095838_110000_CN_317157140_110000/LConn2 -- ВЛ_110_кВ_ПС_Школьная___ПС_Рудянка_CN_275095838_110000_CN_276394749_110000/LConn2
  ВЛ_110_кВ_СУГРЭС___ПС_Школьная_CN_275095838_110000_CN_37479179_110000/LConn3 -- T_275095838_110000;10000_Школьная/LConn3 -- ВЛ_110_кВ_СУГРЭС___ПС_Школьная_CN_275095838_110000_CN_76449471_110000/LConn3 -- ВЛ_110_кВ_СУГРЭС___ПС_Школьная_CN_275095838_110000_CN_66264428_110000/LConn3 -- ВЛ_110_кВ_СУГРЭС___ПС_Школьная_CN_275095838_110000_CN_131114928_110000/LConn3 -- ВЛ_110_кВ_СУГРЭС___ПС_Школьная_CN_275095838_110000_CN_317157140_110000/LConn3 -- ВЛ_110_кВ_ПС_Школьная___ПС_Рудянка_CN_275095838_110000_CN_276394749_110000/LConn3 -- bus47/LConn1
  T_37479179__УЗХР/LConn1 -- ВЛ_110_кВ_СУГРЭС___ПС_Школьная_CN_275095838_110000_CN_37479179_110000/RConn1
  T_37479179__УЗХР/LConn2 -- ВЛ_110_кВ_СУГРЭС___ПС_Школьная_CN_275095838_110000_CN_37479179_110000/RConn2
  ВЛ_110_кВ_СУГРЭС___ПС_Школьная_CN_275095838_110000_CN_37479179_110000/RConn3 -- T_37479179__УЗХР/LConn3 -- bus48/LConn1
  T_76449471_110000;10000_ПС_«Веер»/LConn1 -- ВЛ_110_кВ_СУГРЭС___ПС_Школьная_CN_275095838_110000_CN_76449471_110000/RConn1
  T_76449471_110000;10000_ПС_«Веер»/LConn2 -- ВЛ_110_кВ_СУГРЭС___ПС_Школьная_CN_275095838_110000_CN_76449471_110000/RConn2
  ВЛ_110_кВ_СУГРЭС___ПС_Школьная_CN_275095838_110000_CN_76449471_110000/RConn3 -- T_76449471_110000;10000_ПС_«Веер»/LConn3 -- bus49/LConn1
  T_66264428__Среднеуральская/LConn1 -- ВЛ_110_кВ_СУГРЭС___ПС_Школьная_CN_275095838_110000_CN_66264428_110000/RConn1
  T_66264428__Среднеуральская/LConn2 -- ВЛ_110_кВ_СУГРЭС___ПС_Школьная_CN_275095838_110000_CN_66264428_110000/RConn2
  ВЛ_110_кВ_СУГРЭС___ПС_Школьная_CN_275095838_110000_CN_66264428_110000/RConn3 -- T_66264428__Среднеуральская/LConn3 -- bus50/LConn1
  T_131114928__Термическая/LConn1 -- ВЛ_110_кВ_СУГРЭС___ПС_Школьная_CN_275095838_110000_CN_131114928_110000/RConn1
  T_131114928__Термическая/LConn2 -- ВЛ_110_кВ_СУГРЭС___ПС_Школьная_CN_275095838_110000_CN_131114928_110000/RConn2
  ВЛ_110_кВ_СУГРЭС___ПС_Школьная_CN_275095838_110000_CN_131114928_110000/RConn3 -- T_131114928__Термическая/LConn3 -- bus51/LConn1
  T_317157140_110000;6000_ПС_Электромедь/LConn1 -- ВЛ_110_кВ_СУГРЭС___ПС_Школьная_CN_275095838_110000_CN_317157140_110000/RConn1
  T_317157140_110000;6000_ПС_Электромедь/LConn2 -- ВЛ_110_кВ_СУГРЭС___ПС_Школьная_CN_275095838_110000_CN_317157140_110000/RConn2
  ВЛ_110_кВ_СУГРЭС___ПС_Школьная_CN_275095838_110000_CN_317157140_110000/RConn3 -- T_317157140_110000;6000_ПС_Электромедь/LConn3 -- bus52/LConn1
  ВЛ_110_кВ_ПС_Школьная___ПС_Рудянка_CN_275095838_110000_CN_276394749_110000/RConn1 -- T_276394749_110000;6000_ПС_Рудянка/LConn1 -- ВЛ_110_кВ_ВТГРЭС___ПС_Рудянка_CN_276394749_110000_CN_188857424_110000/LConn1
  ВЛ_110_кВ_ПС_Школьная___ПС_Рудянка_CN_275095838_110000_CN_276394749_110000/RConn2 -- T_276394749_110000;6000_ПС_Рудянка/LConn2 -- ВЛ_110_кВ_ВТГРЭС___ПС_Рудянка_CN_276394749_110000_CN_188857424_110000/LConn2
  ВЛ_110_кВ_ПС_Школьная___ПС_Рудянка_CN_275095838_110000_CN_276394749_110000/RConn3 -- T_276394749_110000;6000_ПС_Рудянка/LConn3 -- ВЛ_110_кВ_ВТГРЭС___ПС_Рудянка_CN_276394749_110000_CN_188857424_110000/LConn3 -- bus53/LConn1
  T_273707087__ГПП_«Солнечная»/LConn1 -- ВЛ_110_кВ_Окунево___Солнечная_1_CN_273707087_110000_CN_110538007_110000/LConn1
  T_273707087__ГПП_«Солнечная»/LConn2 -- ВЛ_110_кВ_Окунево___Солнечная_1_CN_273707087_110000_CN_110538007_110000/LConn2
  ВЛ_110_кВ_Окунево___Солнечная_1_CN_273707087_110000_CN_110538007_110000/LConn3 -- T_273707087__ГПП_«Солнечная»/LConn3 -- bus54/LConn1
  T_110538007_220000;110000;35000_ПС_«Окунево»/LConn1 -- ВЛ_110_кВ_Окунево___Солнечная_1_CN_273707087_110000_CN_110538007_110000/RConn1
  T_110538007_220000;110000;35000_ПС_«Окунево»/LConn2 -- ВЛ_110_кВ_Окунево___Солнечная_1_CN_273707087_110000_CN_110538007_110000/RConn2
  ВЛ_110_кВ_Окунево___Солнечная_1_CN_273707087_110000_CN_110538007_110000/RConn3 -- T_110538007_220000;110000;35000_ПС_«Окунево»/LConn3 -- bus55/LConn1
  T_250194000__ПС_Арси/LConn1 -- ВЛ_110кВ_Кр_Горка_Арси_CN_250194000_110000_CN_191446930_110000/LConn1
  T_250194000__ПС_Арси/LConn2 -- ВЛ_110кВ_Кр_Горка_Арси_CN_250194000_110000_CN_191446930_110000/LConn2
  ВЛ_110кВ_Кр_Горка_Арси_CN_250194000_110000_CN_191446930_110000/LConn3 -- T_250194000__ПС_Арси/LConn3 -- bus56/LConn1
  ВЛ_110кВ_Кр_Горка_Арси_CN_250194000_110000_CN_191446930_110000/RConn1 -- T_191446930__Подстанция/LConn1 -- ВЛ_110кВ_Кр_Горка_Березинская_CN_314008364_110000_CN_191446930_110000/LConn1 -- ВЛ_110кВ_ПС90_Кр_Горка_отпайка_на_Фершампенуаз_CN_199389117_110000_CN_191446930_110000/LConn1
  ВЛ_110кВ_Кр_Горка_Арси_CN_250194000_110000_CN_191446930_110000/RConn2 -- T_191446930__Подстанция/LConn2 -- ВЛ_110кВ_Кр_Горка_Березинская_CN_314008364_110000_CN_191446930_110000/LConn2 -- ВЛ_110кВ_ПС90_Кр_Горка_отпайка_на_Фершампенуаз_CN_199389117_110000_CN_191446930_110000/LConn2
  ВЛ_110кВ_Кр_Горка_Арси_CN_250194000_110000_CN_191446930_110000/RConn3 -- T_191446930__Подстанция/LConn3 -- ВЛ_110кВ_Кр_Горка_Березинская_CN_314008364_110000_CN_191446930_110000/LConn3 -- bus57/LConn1 -- ВЛ_110кВ_ПС90_Кр_Горка_отпайка_на_Фершампенуаз_CN_199389117_110000_CN_191446930_110000/LConn3
  _CN_139662419_110000_CN_165574395_110000/LConn1 -- T_139662419_110000_/LConn1 -- _CN_139662419_110000_CN_26354372_110000/LConn1
  _CN_139662419_110000_CN_165574395_110000/LConn2 -- T_139662419_110000_/LConn2 -- _CN_139662419_110000_CN_26354372_110000/LConn2
  _CN_139662419_110000_CN_165574395_110000/LConn3 -- T_139662419_110000_/LConn3 -- _CN_139662419_110000_CN_26354372_110000/LConn3 -- bus58/LConn1
  T_165574395_110000_Таганай/LConn1 -- _CN_139662419_110000_CN_165574395_110000/RConn1
  T_165574395_110000_Таганай/LConn2 -- _CN_139662419_110000_CN_165574395_110000/RConn2
  _CN_139662419_110000_CN_165574395_110000/RConn3 -- T_165574395_110000_Таганай/LConn3 -- bus59/LConn1
  _CN_139662419_110000_CN_26354372_110000/RConn1 -- T_26354372_110000_Миасс/LConn1 -- _CN_144437268_110000_CN_26354372_110000/LConn1
  _CN_139662419_110000_CN_26354372_110000/RConn2 -- T_26354372_110000_Миасс/LConn2 -- _CN_144437268_110000_CN_26354372_110000/LConn2
  _CN_139662419_110000_CN_26354372_110000/RConn3 -- T_26354372_110000_Миасс/LConn3 -- _CN_144437268_110000_CN_26354372_110000/LConn3 -- bus60/LConn1
  T_99731541__/LConn1 -- _CN_99731541_110000_CN_101747976_110000/LConn1
  T_99731541__/LConn2 -- _CN_99731541_110000_CN_101747976_110000/LConn2
  _CN_99731541_110000_CN_101747976_110000/LConn3 -- T_99731541__/LConn3 -- bus61/LConn1
  _CN_99731541_110000_CN_101747976_110000/RConn1 -- T_101747976__/LConn1 -- _CN_101747976_110000_CN_111353172_110000/LConn1
  _CN_99731541_110000_CN_101747976_110000/RConn2 -- T_101747976__/LConn2 -- _CN_101747976_110000_CN_111353172_110000/LConn2
  _CN_99731541_110000_CN_101747976_110000/RConn3 -- T_101747976__/LConn3 -- _CN_101747976_110000_CN_111353172_110000/LConn3 -- bus62/LConn1
  _CN_99875927_110000_CN_101594027_110000/LConn1 -- T_99875927__/LConn1 -- _CN_99875927_110000_CN_99869836_110000/LConn1
  _CN_99875927_110000_CN_101594027_110000/LConn2 -- T_99875927__/LConn2 -- _CN_99875927_110000_CN_99869836_110000/LConn2
  _CN_99875927_110000_CN_101594027_110000/LConn3 -- T_99875927__/LConn3 -- _CN_99875927_110000_CN_99869836_110000/LConn3 -- bus63/LConn1
  T_101594027__/LConn1 -- _CN_99875927_110000_CN_101594027_110000/RConn1
  T_101594027__/LConn2 -- _CN_99875927_110000_CN_101594027_110000/RConn2
  _CN_99875927_110000_CN_101594027_110000/RConn3 -- T_101594027__/LConn3 -- bus64/LConn1
  T_99869836__Бульварная/LConn1 -- _CN_99875927_110000_CN_99869836_110000/RConn1
  T_99869836__Бульварная/LConn2 -- _CN_99875927_110000_CN_99869836_110000/RConn2
  _CN_99875927_110000_CN_99869836_110000/RConn3 -- T_99869836__Бульварная/LConn3 -- bus65/LConn1
  T_361266572_110000_Гранит/LConn1 -- _CN_361266572_110000_CN_116299140_110000/RConn1
  T_361266572_110000_Гранит/LConn2 -- _CN_361266572_110000_CN_116299140_110000/RConn2
  _CN_361266572_110000_CN_116299140_110000/RConn3 -- T_361266572_110000_Гранит/LConn3 -- bus66/LConn1
  T_117325672__ПС_Пивкино_Тяга_110_10/LConn1 -- _CN_115981920_110000_CN_117325672_110000/RConn1
  T_117325672__ПС_Пивкино_Тяга_110_10/LConn2 -- _CN_115981920_110000_CN_117325672_110000/RConn2
  _CN_115981920_110000_CN_117325672_110000/RConn3 -- T_117325672__ПС_Пивкино_Тяга_110_10/LConn3 -- bus67/LConn1
  T_117325678__ПС_Алакуль_Тяга_110_10/LConn1 -- _CN_115981920_110000_CN_117325678_110000/RConn1
  T_117325678__ПС_Алакуль_Тяга_110_10/LConn2 -- _CN_115981920_110000_CN_117325678_110000/RConn2
  _CN_115981920_110000_CN_117325678_110000/RConn3 -- T_117325678__ПС_Алакуль_Тяга_110_10/LConn3 -- bus68/LConn1
  T_106889826__/LConn1 -- _CN_106889826_110000_CN_41528780_110000/LConn1
  T_106889826__/LConn2 -- _CN_106889826_110000_CN_41528780_110000/LConn2
  _CN_106889826_110000_CN_41528780_110000/LConn3 -- T_106889826__/LConn3 -- bus69/LConn1
  _CN_106889826_110000_CN_41528780_110000/RConn1 -- T_41528780_500000_Подстанция_500_кВ___Златоуст/RConn1 -- L_41528780/LConn1
  _CN_106889826_110000_CN_41528780_110000/RConn2 -- T_41528780_500000_Подстанция_500_кВ___Златоуст/RConn2 -- L_41528780/LConn2
  _CN_106889826_110000_CN_41528780_110000/RConn3 -- T_41528780_500000_Подстанция_500_кВ___Златоуст/RConn3 -- L_41528780/LConn3 -- bus70/LConn1
  T_235846243_110000;6000_ПС_Першино/LConn1 -- ВЛ_110_кВ_ПС_Черемухово___ПС_Першино_CN_235846243_110000_CN_281707739_110000/LConn1
  T_235846243_110000;6000_ПС_Першино/LConn2 -- ВЛ_110_кВ_ПС_Черемухово___ПС_Першино_CN_235846243_110000_CN_281707739_110000/LConn2
  ВЛ_110_кВ_ПС_Черемухово___ПС_Першино_CN_235846243_110000_CN_281707739_110000/LConn3 -- T_235846243_110000;6000_ПС_Першино/LConn3 -- bus71/LConn1
  T_281707739_110000;35000;6000_ПС_Черёмухово/LConn1 -- ВЛ_110_кВ_ПС_Черемухово___ПС_Першино_CN_235846243_110000_CN_281707739_110000/RConn1
  T_281707739_110000;35000;6000_ПС_Черёмухово/LConn2 -- ВЛ_110_кВ_ПС_Черемухово___ПС_Першино_CN_235846243_110000_CN_281707739_110000/RConn2
  ВЛ_110_кВ_ПС_Черемухово___ПС_Першино_CN_235846243_110000_CN_281707739_110000/RConn3 -- T_281707739_110000;35000;6000_ПС_Черёмухово/LConn3 -- bus72/LConn1
  _CN_182904423_110000_CN_230206278_110000/LConn1 -- T_182904423__/LConn1 -- _CN_182904423_110000_CN_225283934_110000/LConn1
  _CN_182904423_110000_CN_230206278_110000/LConn2 -- T_182904423__/LConn2 -- _CN_182904423_110000_CN_225283934_110000/LConn2
  _CN_182904423_110000_CN_230206278_110000/LConn3 -- T_182904423__/LConn3 -- _CN_182904423_110000_CN_225283934_110000/LConn3 -- bus73/LConn1
  T_230206278__/LConn1 -- _CN_182904423_110000_CN_230206278_110000/RConn1
  T_230206278__/LConn2 -- _CN_182904423_110000_CN_230206278_110000/RConn2
  _CN_182904423_110000_CN_230206278_110000/RConn3 -- T_230206278__/LConn3 -- bus74/LConn1
  T_225283934__Электроподстанция/LConn1 -- _CN_182904423_110000_CN_225283934_110000/RConn1
  T_225283934__Электроподстанция/LConn2 -- _CN_182904423_110000_CN_225283934_110000/RConn2
  _CN_182904423_110000_CN_225283934_110000/RConn3 -- T_225283934__Электроподстанция/LConn3 -- bus75/LConn1
  ВЛ_110_кВ_ПС_Юшала___ПС_Яр_CN_200241256_110000_CN_279664560_110000/LConn1 -- T_200241256_110000;10000_ПС_Яр/LConn1 -- ВЛ_110_кВ_ПС_Яр___ПС_Истоур_CN_200241256_110000_CN_280145603_110000/LConn1
  ВЛ_110_кВ_ПС_Юшала___ПС_Яр_CN_200241256_110000_CN_279664560_110000/LConn2 -- T_200241256_110000;10000_ПС_Яр/LConn2 -- ВЛ_110_кВ_ПС_Яр___ПС_Истоур_CN_200241256_110000_CN_280145603_110000/LConn2
  ВЛ_110_кВ_ПС_Юшала___ПС_Яр_CN_200241256_110000_CN_279664560_110000/LConn3 -- T_200241256_110000;10000_ПС_Яр/LConn3 -- ВЛ_110_кВ_ПС_Яр___ПС_Истоур_CN_200241256_110000_CN_280145603_110000/LConn3 -- bus76/LConn1
  T_279664560_110000;10000_ПС_Юшала/LConn1 -- ВЛ_110_кВ_ПС_Юшала___ПС_Яр_CN_200241256_110000_CN_279664560_110000/RConn1
  T_279664560_110000;10000_ПС_Юшала/LConn2 -- ВЛ_110_кВ_ПС_Юшала___ПС_Яр_CN_200241256_110000_CN_279664560_110000/RConn2
  ВЛ_110_кВ_ПС_Юшала___ПС_Яр_CN_200241256_110000_CN_279664560_110000/RConn3 -- T_279664560_110000;10000_ПС_Юшала/LConn3 -- bus77/LConn1
  T_280145603_110000;10000_ПС_Истоур/LConn1 -- ВЛ_110_кВ_ПС_Яр___ПС_Истоур_CN_200241256_110000_CN_280145603_110000/RConn1
  T_280145603_110000;10000_ПС_Истоур/LConn2 -- ВЛ_110_кВ_ПС_Яр___ПС_Истоур_CN_200241256_110000_CN_280145603_110000/RConn2
  ВЛ_110_кВ_ПС_Яр___ПС_Истоур_CN_200241256_110000_CN_280145603_110000/RConn3 -- T_280145603_110000;10000_ПС_Истоур/LConn3 -- bus78/LConn1
  T_114780778__Новоградская/LConn1 -- _CN_114780778_110000_CN_100306689_110000/LConn1
  T_114780778__Новоградская/LConn2 -- _CN_114780778_110000_CN_100306689_110000/LConn2
  _CN_114780778_110000_CN_100306689_110000/LConn3 -- T_114780778__Новоградская/LConn3 -- bus79/LConn1
  T_100306689__Спортивная/LConn1 -- _CN_114780778_110000_CN_100306689_110000/RConn1
  T_100306689__Спортивная/LConn2 -- _CN_114780778_110000_CN_100306689_110000/RConn2
  _CN_114780778_110000_CN_100306689_110000/RConn3 -- T_100306689__Спортивная/LConn3 -- bus80/LConn1
  ВЛ_110кВ_ПС90_Кр_Горка_отпайка_на_Фершампенуаз_CN_199389117_110000_CN_191446930_110000/RConn1 -- T_199389117__Подстанция/LConn1 -- ВЛ_110кВ_ПС90_Кр_Горка_отпайка_на_Фершампенуаз_CN_199389117_110000_CN_339193644_110000/LConn1
  ВЛ_110кВ_ПС90_Кр_Горка_отпайка_на_Фершампенуаз_CN_199389117_110000_CN_191446930_110000/RConn2 -- T_199389117__Подстанция/LConn2 -- ВЛ_110кВ_ПС90_Кр_Горка_отпайка_на_Фершампенуаз_CN_199389117_110000_CN_339193644_110000/LConn2
  ВЛ_110кВ_ПС90_Кр_Горка_отпайка_на_Фершампенуаз_CN_199389117_110000_CN_191446930_110000/RConn3 -- T_199389117__Подстанция/LConn3 -- ВЛ_110кВ_ПС90_Кр_Горка_отпайка_на_Фершампенуаз_CN_199389117_110000_CN_339193644_110000/LConn3 -- bus81/LConn1
  T_339193644__/LConn1 -- ВЛ_110кВ_ПС90_Кр_Горка_отпайка_на_Фершампенуаз_CN_199389117_110000_CN_339193644_110000/RConn1
  T_339193644__/LConn2 -- ВЛ_110кВ_ПС90_Кр_Горка_отпайка_на_Фершампенуаз_CN_199389117_110000_CN_339193644_110000/RConn2
  ВЛ_110кВ_ПС90_Кр_Горка_отпайка_на_Фершампенуаз_CN_199389117_110000_CN_339193644_110000/RConn3 -- T_339193644__/LConn3 -- bus82/LConn1
  T_118008950__/LConn1 -- _CN_118008950_110000_CN_117941010_110000/LConn1
  T_118008950__/LConn2 -- _CN_118008950_110000_CN_117941010_110000/LConn2
  _CN_118008950_110000_CN_117941010_110000/LConn3 -- T_118008950__/LConn3 -- bus83/LConn1
  _CN_118008950_110000_CN_117941010_110000/RConn1 -- T_117941010__ПС_Чудиново_110_10/LConn1 -- _CN_117941027_110000_CN_117941010_110000/LConn1
  _CN_118008950_110000_CN_117941010_110000/RConn2 -- T_117941010__ПС_Чудиново_110_10/LConn2 -- _CN_117941027_110000_CN_117941010_110000/LConn2
  _CN_118008950_110000_CN_117941010_110000/RConn3 -- T_117941010__ПС_Чудиново_110_10/LConn3 -- _CN_117941027_110000_CN_117941010_110000/LConn3 -- bus84/LConn1
  _CN_144437268_110000_CN_189890975_110000/RConn1 -- T_144437268__Автозаводская/LConn1 -- _CN_144437268_110000_CN_26354372_110000/RConn1
  _CN_144437268_110000_CN_189890975_110000/RConn2 -- T_144437268__Автозаводская/LConn2 -- _CN_144437268_110000_CN_26354372_110000/RConn2
  _CN_144437268_110000_CN_189890975_110000/RConn3 -- T_144437268__Автозаводская/LConn3 -- _CN_144437268_110000_CN_26354372_110000/RConn3 -- bus85/LConn1
  ПС_Таволги___ПС_Киприно___ПС_Черемисска_CN_273461546_110000_CN_273649961_110000/LConn1 -- T_273461546_110000;10000_ПС_Киприно/LConn1 -- ПС_Таволги___ПС_Киприно___ПС_Черемисска_CN_273461546_110000_CN_101532642_110000/LConn1 -- ПС_Таволги___ПС_Киприно___ПС_Черемисска_CN_273461546_110000_CN_135780398_110000/LConn1
  ПС_Таволги___ПС_Киприно___ПС_Черемисска_CN_273461546_110000_CN_273649961_110000/LConn2 -- T_273461546_110000;10000_ПС_Киприно/LConn2 -- ПС_Таволги___ПС_Киприно___ПС_Черемисска_CN_273461546_110000_CN_101532642_110000/LConn2 -- ПС_Таволги___ПС_Киприно___ПС_Черемисска_CN_273461546_110000_CN_135780398_110000/LConn2
  ПС_Таволги___ПС_Киприно___ПС_Черемисска_CN_273461546_110000_CN_273649961_110000/LConn3 -- T_273461546_110000;10000_ПС_Киприно/LConn3 -- ПС_Таволги___ПС_Киприно___ПС_Черемисска_CN_273461546_110000_CN_101532642_110000/LConn3 -- ПС_Таволги___ПС_Киприно___ПС_Черемисска_CN_273461546_110000_CN_135780398_110000/LConn3 -- bus86/LConn1
  T_273649961_110000;35000;10000_ПС_Черемисска/LConn1 -- ПС_Таволги___ПС_Киприно___ПС_Черемисска_CN_273461546_110000_CN_273649961_110000/RConn1
  T_273649961_110000;35000;10000_ПС_Черемисска/LConn2 -- ПС_Таволги___ПС_Киприно___ПС_Черемисска_CN_273461546_110000_CN_273649961_110000/RConn2
  ПС_Таволги___ПС_Киприно___ПС_Черемисска_CN_273461546_110000_CN_273649961_110000/RConn3 -- T_273649961_110000;35000;10000_ПС_Черемисска/LConn3 -- bus87/LConn1
  T_101532642_110000;35000;10000_ПС_Таволги/LConn1 -- ПС_Таволги___ПС_Киприно___ПС_Черемисска_CN_273461546_110000_CN_101532642_110000/RConn1
  T_101532642_110000;35000;10000_ПС_Таволги/LConn2 -- ПС_Таволги___ПС_Киприно___ПС_Черемисска_CN_273461546_110000_CN_101532642_110000/RConn2
  ПС_Таволги___ПС_Киприно___ПС_Черемисска_CN_273461546_110000_CN_101532642_110000/RConn3 -- T_101532642_110000;35000;10000_ПС_Таволги/LConn3 -- bus88/LConn1
  T_135780398__/LConn1 -- ПС_Таволги___ПС_Киприно___ПС_Черемисска_CN_273461546_110000_CN_135780398_110000/RConn1
  T_135780398__/LConn2 -- ПС_Таволги___ПС_Киприно___ПС_Черемисска_CN_273461546_110000_CN_135780398_110000/RConn2
  ПС_Таволги___ПС_Киприно___ПС_Черемисска_CN_273461546_110000_CN_135780398_110000/RConn3 -- T_135780398__/LConn3 -- bus89/LConn1
  T_306102396__/LConn1 -- _CN_306102396_110000_CN_305096727_110000/LConn1
  T_306102396__/LConn2 -- _CN_306102396_110000_CN_305096727_110000/LConn2
  _CN_306102396_110000_CN_305096727_110000/LConn3 -- T_306102396__/LConn3 -- bus90/LConn1
  _CN_306102396_110000_CN_305096727_110000/RConn1 -- T_305096727__/LConn1 -- _CN_305096727_110000_CN_354777580_110000/LConn1
  _CN_306102396_110000_CN_305096727_110000/RConn2 -- T_305096727__/LConn2 -- _CN_305096727_110000_CN_354777580_110000/LConn2
  _CN_306102396_110000_CN_305096727_110000/RConn3 -- T_305096727__/LConn3 -- _CN_305096727_110000_CN_354777580_110000/LConn3 -- bus91/LConn1
  _CN_117325674_110000_CN_117941027_110000/RConn1 -- T_117941027__ПС_Сулейманово_110_35_10/LConn1 -- _CN_117941027_110000_CN_117941010_110000/RConn1
  _CN_117325674_110000_CN_117941027_110000/RConn2 -- T_117941027__ПС_Сулейманово_110_35_10/LConn2 -- _CN_117941027_110000_CN_117941010_110000/RConn2
  _CN_117325674_110000_CN_117941027_110000/RConn3 -- T_117941027__ПС_Сулейманово_110_35_10/LConn3 -- _CN_117941027_110000_CN_117941010_110000/RConn3 -- bus92/LConn1
  T_104952455__ПС_Уфалей/LConn1 -- _CN_104952455_110000_CN_196250439_110000/LConn1
  T_104952455__ПС_Уфалей/LConn2 -- _CN_104952455_110000_CN_196250439_110000/LConn2
  _CN_104952455_110000_CN_196250439_110000/LConn3 -- T_104952455__ПС_Уфалей/LConn3 -- bus93/LConn1
  T_196250439__/LConn1 -- _CN_104952455_110000_CN_196250439_110000/RConn1
  T_196250439__/LConn2 -- _CN_104952455_110000_CN_196250439_110000/RConn2
  _CN_104952455_110000_CN_196250439_110000/RConn3 -- T_196250439__/LConn3 -- bus94/LConn1
  T_361265069_110000_Мисяш/LConn1 -- _CN_361265069_110000_CN_116299140_110000/RConn1
  T_361265069_110000_Мисяш/LConn2 -- _CN_361265069_110000_CN_116299140_110000/RConn2
  _CN_361265069_110000_CN_116299140_110000/RConn3 -- T_361265069_110000_Мисяш/LConn3 -- bus95/LConn1
  T_266070665__Измоденово/LConn1 -- _CN_266070665_110000_CN_130127057_110000/LConn1
  T_266070665__Измоденово/LConn2 -- _CN_266070665_110000_CN_130127057_110000/LConn2
  _CN_266070665_110000_CN_130127057_110000/LConn3 -- T_266070665__Измоденово/LConn3 -- bus96/LConn1
  T_130127057__/LConn1 -- _CN_266070665_110000_CN_130127057_110000/RConn1
  T_130127057__/LConn2 -- _CN_266070665_110000_CN_130127057_110000/RConn2
  _CN_266070665_110000_CN_130127057_110000/RConn3 -- T_130127057__/LConn3 -- bus97/LConn1
  T_139658378__/LConn1 -- _CN_139658378_110000_CN_139658358_110000/LConn1
  T_139658378__/LConn2 -- _CN_139658378_110000_CN_139658358_110000/LConn2
  _CN_139658378_110000_CN_139658358_110000/LConn3 -- T_139658378__/LConn3 -- bus98/LConn1
  T_139658358__Северная/LConn1 -- _CN_139658378_110000_CN_139658358_110000/RConn1
  T_139658358__Северная/LConn2 -- _CN_139658378_110000_CN_139658358_110000/RConn2
  _CN_139658378_110000_CN_139658358_110000/RConn3 -- T_139658358__Северная/LConn3 -- bus99/LConn1
  _CN_305096727_110000_CN_354777580_110000/RConn1 -- T_354777580__/LConn1 -- _CN_332377360_110000_CN_354777580_110000/LConn1
  _CN_305096727_110000_CN_354777580_110000/RConn2 -- T_354777580__/LConn2 -- _CN_332377360_110000_CN_354777580_110000/LConn2
  _CN_305096727_110000_CN_354777580_110000/RConn3 -- T_354777580__/LConn3 -- _CN_332377360_110000_CN_354777580_110000/LConn3 -- bus100/LConn1
  T_168166544_110000;fixme_/LConn1 -- _CN_168166544_110000_CN_168174311_110000/LConn1
  T_168166544_110000;fixme_/LConn2 -- _CN_168166544_110000_CN_168174311_110000/LConn2
  _CN_168166544_110000_CN_168174311_110000/LConn3 -- T_168166544_110000;fixme_/LConn3 -- bus101/LConn1
  T_168174311__/LConn1 -- _CN_168166544_110000_CN_168174311_110000/RConn1
  T_168174311__/LConn2 -- _CN_168166544_110000_CN_168174311_110000/RConn2
  _CN_168166544_110000_CN_168174311_110000/RConn3 -- T_168174311__/LConn3 -- bus102/LConn1
  T_105584274_110000;6000_ПС_Черноисточинск/LConn1 -- ВЛ_110_кВ_ПС_Черноисточинск___ПС_НЦЗ_CN_105584274_110000_CN_274851642_110000/LConn1
  T_105584274_110000;6000_ПС_Черноисточинск/LConn2 -- ВЛ_110_кВ_ПС_Черноисточинск___ПС_НЦЗ_CN_105584274_110000_CN_274851642_110000/LConn2
  ВЛ_110_кВ_ПС_Черноисточинск___ПС_НЦЗ_CN_105584274_110000_CN_274851642_110000/LConn3 -- T_105584274_110000;6000_ПС_Черноисточинск/LConn3 -- bus103/LConn1
  T_274851642_110000;6000_ПС_НЦЗ/LConn1 -- ВЛ_110_кВ_ПС_Черноисточинск___ПС_НЦЗ_CN_105584274_110000_CN_274851642_110000/RConn1
  T_274851642_110000;6000_ПС_НЦЗ/LConn2 -- ВЛ_110_кВ_ПС_Черноисточинск___ПС_НЦЗ_CN_105584274_110000_CN_274851642_110000/RConn2
  ВЛ_110_кВ_ПС_Черноисточинск___ПС_НЦЗ_CN_105584274_110000_CN_274851642_110000/RConn3 -- T_274851642_110000;6000_ПС_НЦЗ/LConn3 -- bus104/LConn1
  _CN_372580506_110000_CN_98423617_110000/RConn1 -- T_98423617_500000_Шагол/RConn4 -- L_98423617/LConn1
  _CN_372580506_110000_CN_98423617_110000/RConn2 -- T_98423617_500000_Шагол/RConn5 -- L_98423617/LConn2
  _CN_372580506_110000_CN_98423617_110000/RConn3 -- T_98423617_500000_Шагол/RConn6 -- L_98423617/LConn3 -- bus105/LConn1
  _CN_361264295_110000_CN_372580522_110000/LConn1 -- T_361264295_110000_Луговая/LConn1 -- _CN_361264295_110000_CN_116299140_110000/RConn1
  _CN_361264295_110000_CN_372580522_110000/LConn2 -- T_361264295_110000_Луговая/LConn2 -- _CN_361264295_110000_CN_116299140_110000/RConn2
  _CN_361264295_110000_CN_372580522_110000/LConn3 -- T_361264295_110000_Луговая/LConn3 -- _CN_361264295_110000_CN_116299140_110000/RConn3 -- bus106/LConn1
  T_372580522_110000_Тимирязевская/LConn1 -- _CN_361264295_110000_CN_372580522_110000/RConn1
  T_372580522_110000_Тимирязевская/LConn2 -- _CN_361264295_110000_CN_372580522_110000/RConn2
  _CN_361264295_110000_CN_372580522_110000/RConn3 -- T_372580522_110000_Тимирязевская/LConn3 -- bus107/LConn1
  _CN_97947939_110000_CN_176374151_110000/LConn1 -- T_97947939__ПС_«Загородная»/LConn1 -- _CN_97947939_110000_CN_38919677_110000/LConn1
  _CN_97947939_110000_CN_176374151_110000/LConn2 -- T_97947939__ПС_«Загородная»/LConn2 -- _CN_97947939_110000_CN_38919677_110000/LConn2
  _CN_97947939_110000_CN_176374151_110000/LConn3 -- T_97947939__ПС_«Загородная»/LConn3 -- _CN_97947939_110000_CN_38919677_110000/LConn3 -- bus108/LConn1
  T_176374151__Унипромедь/LConn1 -- _CN_97947939_110000_CN_176374151_110000/RConn1
  T_176374151__Унипромедь/LConn2 -- _CN_97947939_110000_CN_176374151_110000/RConn2
  _CN_97947939_110000_CN_176374151_110000/RConn3 -- T_176374151__Унипромедь/LConn3 -- bus109/LConn1
  T_38919677__Сибирская/LConn1 -- _CN_97947939_110000_CN_38919677_110000/RConn1
  T_38919677__Сибирская/LConn2 -- _CN_97947939_110000_CN_38919677_110000/RConn2
  _CN_97947939_110000_CN_38919677_110000/RConn3 -- T_38919677__Сибирская/LConn3 -- bus110/LConn1
  ВЛ_110_кВ_ВТГРЭС___ПС_Рудянка_CN_276394749_110000_CN_188857424_110000/RConn1 -- G_188857424_Верхнетагильская_ГРЭС/RConn1 -- Отпайка_ВЛ_110_кВ_на_ПС_Твёрдые_сплавы_от_ВТГРЭС___Карпушиха_CN_276394758_110000_CN_188857424_110000/LConn1
  ВЛ_110_кВ_ВТГРЭС___ПС_Рудянка_CN_276394749_110000_CN_188857424_110000/RConn2 -- G_188857424_Верхнетагильская_ГРЭС/RConn2 -- Отпайка_ВЛ_110_кВ_на_ПС_Твёрдые_сплавы_от_ВТГРЭС___Карпушиха_CN_276394758_110000_CN_188857424_110000/LConn2
  ВЛ_110_кВ_ВТГРЭС___ПС_Рудянка_CN_276394749_110000_CN_188857424_110000/RConn3 -- G_188857424_Верхнетагильская_ГРЭС/RConn3 -- Отпайка_ВЛ_110_кВ_на_ПС_Твёрдые_сплавы_от_ВТГРЭС___Карпушиха_CN_276394758_110000_CN_188857424_110000/LConn3 -- bus111/LConn1
  T_352282301_110000_Тумак/LConn1 -- _CN_352282301_110000_CN_138410290_110000/LConn1
  T_352282301_110000_Тумак/LConn2 -- _CN_352282301_110000_CN_138410290_110000/LConn2
  _CN_352282301_110000_CN_138410290_110000/LConn3 -- T_352282301_110000_Тумак/LConn3 -- bus112/LConn1
  T_138410290_110000_Варна/LConn1 -- _CN_352282301_110000_CN_138410290_110000/RConn1
  T_138410290_110000_Варна/LConn2 -- _CN_352282301_110000_CN_138410290_110000/RConn2
  _CN_352282301_110000_CN_138410290_110000/RConn3 -- T_138410290_110000_Варна/LConn3 -- bus113/LConn1
  T_190450368_110000_Подстанция_«Григорьевская»/LConn1 -- _CN_190450368_110000_CN_89555905_110000/LConn1
  T_190450368_110000_Подстанция_«Григорьевская»/LConn2 -- _CN_190450368_110000_CN_89555905_110000/LConn2
  _CN_190450368_110000_CN_89555905_110000/LConn3 -- T_190450368_110000_Подстанция_«Григорьевская»/LConn3 -- bus114/LConn1
  T_89555905_110000_Подстанция_«Стрежевская»/LConn1 -- _CN_190450368_110000_CN_89555905_110000/RConn1
  T_89555905_110000_Подстанция_«Стрежевская»/LConn2 -- _CN_190450368_110000_CN_89555905_110000/RConn2
  _CN_190450368_110000_CN_89555905_110000/RConn3 -- T_89555905_110000_Подстанция_«Стрежевская»/LConn3 -- bus115/LConn1
  T_325873379__/LConn1 -- _CN_325873379_110000_CN_90797306_110000/LConn1
  T_325873379__/LConn2 -- _CN_325873379_110000_CN_90797306_110000/LConn2
  _CN_325873379_110000_CN_90797306_110000/LConn3 -- T_325873379__/LConn3 -- bus116/LConn1
  T_90797306__/LConn1 -- _CN_325873379_110000_CN_90797306_110000/RConn1
  T_90797306__/LConn2 -- _CN_325873379_110000_CN_90797306_110000/RConn2
  _CN_325873379_110000_CN_90797306_110000/RConn3 -- T_90797306__/LConn3 -- bus117/LConn1
  T_130534123__/LConn1 -- _CN_130534123_110000_CN_94087563_110000/LConn1
  T_130534123__/LConn2 -- _CN_130534123_110000_CN_94087563_110000/LConn2
  _CN_130534123_110000_CN_94087563_110000/LConn3 -- T_130534123__/LConn3 -- bus118/LConn1
  _CN_130534123_110000_CN_94087563_110000/RConn1 -- T_94087563__Подстанция_Мегион/RConn1 -- L_94087563/LConn1
  _CN_130534123_110000_CN_94087563_110000/RConn2 -- T_94087563__Подстанция_Мегион/RConn2 -- L_94087563/LConn2
  _CN_130534123_110000_CN_94087563_110000/RConn3 -- T_94087563__Подстанция_Мегион/RConn3 -- L_94087563/LConn3 -- bus119/LConn1
  T_373906159_110000_Княженская/LConn1 -- ВЛ_110_кВ_Новогеоргиевская___Княженская_CN_373906159_110000_CN_144699678_110000/LConn1
  T_373906159_110000_Княженская/LConn2 -- ВЛ_110_кВ_Новогеоргиевская___Княженская_CN_373906159_110000_CN_144699678_110000/LConn2
  ВЛ_110_кВ_Новогеоргиевская___Княженская_CN_373906159_110000_CN_144699678_110000/LConn3 -- T_373906159_110000_Княженская/LConn3 -- bus120/LConn1
  T_144699678_110000_Новогеоргиевская/LConn1 -- ВЛ_110_кВ_Новогеоргиевская___Княженская_CN_373906159_110000_CN_144699678_110000/RConn1
  T_144699678_110000_Новогеоргиевская/LConn2 -- ВЛ_110_кВ_Новогеоргиевская___Княженская_CN_373906159_110000_CN_144699678_110000/RConn2
  ВЛ_110_кВ_Новогеоргиевская___Княженская_CN_373906159_110000_CN_144699678_110000/RConn3 -- T_144699678_110000_Новогеоргиевская/LConn3 -- bus121/LConn1
  _CN_114429183_110000_CN_166629221_110000/LConn1 -- T_114429183__ПС_Первоуральская/LConn1 -- _CN_114429183_110000_CN_212739375_110000/LConn1 -- _CN_114429183_110000_CN_119306741_110000/LConn1
  _CN_114429183_110000_CN_166629221_110000/LConn2 -- T_114429183__ПС_Первоуральская/LConn2 -- _CN_114429183_110000_CN_212739375_110000/LConn2 -- _CN_114429183_110000_CN_119306741_110000/LConn2
  _CN_114429183_110000_CN_166629221_110000/LConn3 -- T_114429183__ПС_Первоуральская/LConn3 -- _CN_114429183_110000_CN_212739375_110000/LConn3 -- _CN_114429183_110000_CN_119306741_110000/LConn3 -- bus122/LConn1
  T_166629221__/LConn1 -- _CN_114429183_110000_CN_166629221_110000/RConn1
  T_166629221__/LConn2 -- _CN_114429183_110000_CN_166629221_110000/RConn2
  _CN_114429183_110000_CN_166629221_110000/RConn3 -- T_166629221__/LConn3 -- bus123/LConn1
  T_212739375__/LConn1 -- _CN_114429183_110000_CN_212739375_110000/RConn1
  T_212739375__/LConn2 -- _CN_114429183_110000_CN_212739375_110000/RConn2
  _CN_114429183_110000_CN_212739375_110000/RConn3 -- T_212739375__/LConn3 -- bus124/LConn1
  T_119306741__/LConn1 -- _CN_114429183_110000_CN_119306741_110000/RConn1
  T_119306741__/LConn2 -- _CN_114429183_110000_CN_119306741_110000/RConn2
  _CN_114429183_110000_CN_119306741_110000/RConn3 -- T_119306741__/LConn3 -- bus125/LConn1
  T_276394758_110000;6000_Твёрдые_сплавы/LConn1 -- Отпайка_ВЛ_110_кВ_на_ПС_Твёрдые_сплавы_от_ВТГРЭС___Карпушиха_CN_276394758_110000_CN_188857424_110000/RConn1
  T_276394758_110000;6000_Твёрдые_сплавы/LConn2 -- Отпайка_ВЛ_110_кВ_на_ПС_Твёрдые_сплавы_от_ВТГРЭС___Карпушиха_CN_276394758_110000_CN_188857424_110000/RConn2
  Отпайка_ВЛ_110_кВ_на_ПС_Твёрдые_сплавы_от_ВТГРЭС___Карпушиха_CN_276394758_110000_CN_188857424_110000/RConn3 -- T_276394758_110000;6000_Твёрдые_сплавы/LConn3 -- bus126/LConn1
  T_111353172__Заречная/LConn1 -- _CN_101747976_110000_CN_111353172_110000/RConn1
  T_111353172__Заречная/LConn2 -- _CN_101747976_110000_CN_111353172_110000/RConn2
  _CN_101747976_110000_CN_111353172_110000/RConn3 -- T_111353172__Заречная/LConn3 -- bus127/LConn1
  T_332377360__/LConn1 -- _CN_332377360_110000_CN_354777580_110000/RConn1
  T_332377360__/LConn2 -- _CN_332377360_110000_CN_354777580_110000/RConn2
  _CN_332377360_110000_CN_354777580_110000/RConn3 -- T_332377360__/LConn3 -- bus128/LConn1
  T_207569689_110000;35000;6000_ПС_Насосная/LConn1 -- _CN_207569689_110000_CN_95452082_110000/LConn1
  T_207569689_110000;35000;6000_ПС_Насосная/LConn2 -- _CN_207569689_110000_CN_95452082_110000/LConn2
  _CN_207569689_110000_CN_95452082_110000/LConn3 -- T_207569689_110000;35000;6000_ПС_Насосная/LConn3 -- bus129/LConn1
  T_95452082_110000_Даурская/LConn1 -- _CN_207569689_110000_CN_95452082_110000/RConn1
  T_95452082_110000_Даурская/LConn2 -- _CN_207569689_110000_CN_95452082_110000/RConn2
  _CN_207569689_110000_CN_95452082_110000/RConn3 -- T_95452082_110000_Даурская/LConn3 -- bus130/LConn1
  T_229397794_110000;10000_ПС_Тугулым/LConn1 -- ВЛ_110_кВ_ПС_Зарница___ПС_Тугулым_CN_229397794_110000_CN_279664558_110000/LConn1
  T_229397794_110000;10000_ПС_Тугулым/LConn2 -- ВЛ_110_кВ_ПС_Зарница___ПС_Тугулым_CN_229397794_110000_CN_279664558_110000/LConn2
  ВЛ_110_кВ_ПС_Зарница___ПС_Тугулым_CN_229397794_110000_CN_279664558_110000/LConn3 -- T_229397794_110000;10000_ПС_Тугулым/LConn3 -- bus131/LConn1
  T_279664558_110000_ПС_Зарница/LConn1 -- ВЛ_110_кВ_ПС_Зарница___ПС_Тугулым_CN_229397794_110000_CN_279664558_110000/RConn1
  T_279664558_110000_ПС_Зарница/LConn2 -- ВЛ_110_кВ_ПС_Зарница___ПС_Тугулым_CN_229397794_110000_CN_279664558_110000/RConn2
  ВЛ_110_кВ_ПС_Зарница___ПС_Тугулым_CN_229397794_110000_CN_279664558_110000/RConn3 -- T_279664558_110000_ПС_Зарница/LConn3 -- bus132/LConn1
  T_314008364_110000_Березинская/LConn1 -- ВЛ_110кВ_Кр_Горка_Березинская_CN_314008364_110000_CN_191446930_110000/RConn1
  T_314008364_110000_Березинская/LConn2 -- ВЛ_110кВ_Кр_Горка_Березинская_CN_314008364_110000_CN_191446930_110000/RConn2
  ВЛ_110кВ_Кр_Горка_Березинская_CN_314008364_110000_CN_191446930_110000/RConn3 -- T_314008364_110000_Березинская/LConn3 -- bus133/LConn1
  T_282748778__/LConn1 -- _CN_166188874_110000_CN_282748778_110000/RConn1
  T_282748778__/LConn2 -- _CN_166188874_110000_CN_282748778_110000/RConn2
  _CN_166188874_110000_CN_282748778_110000/RConn3 -- T_282748778__/LConn3 -- bus134/LConn1
  T_282850239__/LConn1 -- _CN_166188874_110000_CN_282850239_110000/RConn1
  T_282850239__/LConn2 -- _CN_166188874_110000_CN_282850239_110000/RConn2
  _CN_166188874_110000_CN_282850239_110000/RConn3 -- T_282850239__/LConn3 -- bus135/LConn1
  _CN_166188874_110000_CN_92045303_110000/RConn1 -- T_92045303__/LConn1 -- _CN_282779592_110000_CN_92045303_110000/LConn1
  _CN_166188874_110000_CN_92045303_110000/RConn2 -- T_92045303__/LConn2 -- _CN_282779592_110000_CN_92045303_110000/LConn2
  _CN_166188874_110000_CN_92045303_110000/RConn3 -- T_92045303__/LConn3 -- _CN_282779592_110000_CN_92045303_110000/LConn3 -- bus136/LConn1
  T_255032299__/LConn1 -- _CN_255032299_110000_CN_255032301_110000/LConn1
  T_255032299__/LConn2 -- _CN_255032299_110000_CN_255032301_110000/LConn2
  _CN_255032299_110000_CN_255032301_110000/LConn3 -- T_255032299__/LConn3 -- bus137/LConn1
  T_255032301__/LConn1 -- _CN_255032299_110000_CN_255032301_110000/RConn1
  T_255032301__/LConn2 -- _CN_255032299_110000_CN_255032301_110000/RConn2
  _CN_255032299_110000_CN_255032301_110000/RConn3 -- T_255032301__/LConn3 -- bus138/LConn1
  T_189890976__ОРУ_110_кВ/LConn1 -- _CN_189890975_110000_CN_189890976_110000/RConn1
  T_189890976__ОРУ_110_кВ/LConn2 -- _CN_189890975_110000_CN_189890976_110000/RConn2
  _CN_189890975_110000_CN_189890976_110000/RConn3 -- T_189890976__ОРУ_110_кВ/LConn3 -- bus139/LConn1
  T_279664559_110000_ПС_Кармак/LConn1 -- ВЛ_110_кВ_ПС_Кармак___ПС_Верховино_CN_279664559_110000_CN_174028758_110000/LConn1
  T_279664559_110000_ПС_Кармак/LConn2 -- ВЛ_110_кВ_ПС_Кармак___ПС_Верховино_CN_279664559_110000_CN_174028758_110000/LConn2
  ВЛ_110_кВ_ПС_Кармак___ПС_Верховино_CN_279664559_110000_CN_174028758_110000/LConn3 -- T_279664559_110000_ПС_Кармак/LConn3 -- bus140/LConn1
  ВЛ_110_кВ_ПС_Кармак___ПС_Верховино_CN_279664559_110000_CN_174028758_110000/RConn1 -- T_174028758_110000;10000_ПС_Верховино/LConn1 -- ВЛ_110_кВ_Верховино_Успенка_CN_174028758_110000_CN_277716444_110000/LConn1
  ВЛ_110_кВ_ПС_Кармак___ПС_Верховино_CN_279664559_110000_CN_174028758_110000/RConn2 -- T_174028758_110000;10000_ПС_Верховино/LConn2 -- ВЛ_110_кВ_Верховино_Успенка_CN_174028758_110000_CN_277716444_110000/LConn2
  ВЛ_110_кВ_ПС_Кармак___ПС_Верховино_CN_279664559_110000_CN_174028758_110000/RConn3 -- T_174028758_110000;10000_ПС_Верховино/LConn3 -- ВЛ_110_кВ_Верховино_Успенка_CN_174028758_110000_CN_277716444_110000/LConn3 -- bus141/LConn1
  T_281458614_220000;110000_ПС_Краснотурьинск/LConn1 -- ВЛ_110_кВ_ПС_Краснотурьинск___ПС_Североуральск_CN_281458614_110000_CN_281458615_110000/LConn1
  T_281458614_220000;110000_ПС_Краснотурьинск/LConn2 -- ВЛ_110_кВ_ПС_Краснотурьинск___ПС_Североуральск_CN_281458614_110000_CN_281458615_110000/LConn2
  ВЛ_110_кВ_ПС_Краснотурьинск___ПС_Североуральск_CN_281458614_110000_CN_281458615_110000/LConn3 -- T_281458614_220000;110000_ПС_Краснотурьинск/LConn3 -- bus142/LConn1
  T_281458615_110000;35000;6000_ПС_Североуральск/LConn1 -- ВЛ_110_кВ_ПС_Краснотурьинск___ПС_Североуральск_CN_281458614_110000_CN_281458615_110000/RConn1
  T_281458615_110000;35000;6000_ПС_Североуральск/LConn2 -- ВЛ_110_кВ_ПС_Краснотурьинск___ПС_Североуральск_CN_281458614_110000_CN_281458615_110000/RConn2
  ВЛ_110_кВ_ПС_Краснотурьинск___ПС_Североуральск_CN_281458614_110000_CN_281458615_110000/RConn3 -- T_281458615_110000;35000;6000_ПС_Североуральск/LConn3 -- bus143/LConn1
  T_282779592__/LConn1 -- _CN_282779592_110000_CN_92045303_110000/RConn1
  T_282779592__/LConn2 -- _CN_282779592_110000_CN_92045303_110000/RConn2
  _CN_282779592_110000_CN_92045303_110000/RConn3 -- T_282779592__/LConn3 -- bus144/LConn1
  T_337947383__/LConn1 -- _CN_337947383_110000_CN_220103258_110000/LConn1
  T_337947383__/LConn2 -- _CN_337947383_110000_CN_220103258_110000/LConn2
  _CN_337947383_110000_CN_220103258_110000/LConn3 -- T_337947383__/LConn3 -- bus145/LConn1
  G_220103258_Зауральская_ТЭЦ/RConn1 -- _CN_337947383_110000_CN_220103258_110000/RConn1
  G_220103258_Зауральская_ТЭЦ/RConn2 -- _CN_337947383_110000_CN_220103258_110000/RConn2
  _CN_337947383_110000_CN_220103258_110000/RConn3 -- G_220103258_Зауральская_ТЭЦ/RConn3 -- bus146/LConn1
  T_386978254_110000_Маякская/LConn1 -- _CN_386978254_110000_CN_163401683_110000/RConn1
  T_386978254_110000_Маякская/LConn2 -- _CN_386978254_110000_CN_163401683_110000/RConn2
  _CN_386978254_110000_CN_163401683_110000/RConn3 -- T_386978254_110000_Маякская/LConn3 -- bus147/LConn1
  T_277716444_110000;10000_ПС_Успенка/LConn1 -- ВЛ_110_кВ_Верховино_Успенка_CN_174028758_110000_CN_277716444_110000/RConn1
  T_277716444_110000;10000_ПС_Успенка/LConn2 -- ВЛ_110_кВ_Верховино_Успенка_CN_174028758_110000_CN_277716444_110000/RConn2
  ВЛ_110_кВ_Верховино_Успенка_CN_174028758_110000_CN_277716444_110000/RConn3 -- T_277716444_110000;10000_ПС_Успенка/LConn3 -- bus148/LConn1
  T_108720649__/LConn1 -- _CN_108720649_220000_CN_93464361_220000/LConn1
  T_108720649__/LConn2 -- _CN_108720649_220000_CN_93464361_220000/LConn2
  _CN_108720649_220000_CN_93464361_220000/LConn3 -- T_108720649__/LConn3 -- bus149/LConn1
  T_93464361__Переключательный_пункт_Сосьва/LConn1 -- _CN_108720649_220000_CN_93464361_220000/RConn1
  T_93464361__Переключательный_пункт_Сосьва/LConn2 -- _CN_108720649_220000_CN_93464361_220000/RConn2
  _CN_108720649_220000_CN_93464361_220000/RConn3 -- T_93464361__Переключательный_пункт_Сосьва/LConn3 -- bus150/LConn1
  T_94087563__Подстанция_Мегион/LConn1 -- _CN_94087563_220000_CN_130506016_220000/LConn1
  T_94087563__Подстанция_Мегион/LConn2 -- _CN_94087563_220000_CN_130506016_220000/LConn2
  _CN_94087563_220000_CN_130506016_220000/LConn3 -- T_94087563__Подстанция_Мегион/LConn3 -- bus151/LConn1
  _CN_94087563_220000_CN_130506016_220000/RConn1 -- T_130506016_500000_Подстанция_«Сибирская»/RConn1 -- L_130506016/LConn1
  _CN_94087563_220000_CN_130506016_220000/RConn2 -- T_130506016_500000_Подстанция_«Сибирская»/RConn2 -- L_130506016/LConn2
  _CN_94087563_220000_CN_130506016_220000/RConn3 -- T_130506016_500000_Подстанция_«Сибирская»/RConn3 -- L_130506016/LConn3 -- bus152/LConn1
  T_96989708__/LConn1 -- _CN_96989708_220000_CN_81131204_220000/LConn1
  T_96989708__/LConn2 -- _CN_96989708_220000_CN_81131204_220000/LConn2
  _CN_96989708_220000_CN_81131204_220000/LConn3 -- T_96989708__/LConn3 -- bus153/LConn1
  _CN_96989708_220000_CN_81131204_220000/RConn1 -- T_81131204_500000;220000;110000;35000_ПС_Южная/LConn1 -- _CN_81131204_220000_CN_150165502_220000/LConn1
  _CN_96989708_220000_CN_81131204_220000/RConn2 -- T_81131204_500000;220000;110000;35000_ПС_Южная/LConn2 -- _CN_81131204_220000_CN_150165502_220000/LConn2
  _CN_96989708_220000_CN_81131204_220000/RConn3 -- T_81131204_500000;220000;110000;35000_ПС_Южная/LConn3 -- _CN_81131204_220000_CN_150165502_220000/LConn3 -- bus154/LConn1
  T_275095874_220000_/LConn1 -- _CN_275095874_220000_CN_93314614_220000/LConn1
  T_275095874_220000_/LConn2 -- _CN_275095874_220000_CN_93314614_220000/LConn2
  _CN_275095874_220000_CN_93314614_220000/LConn3 -- T_275095874_220000_/LConn3 -- bus155/LConn1
  _CN_275095874_220000_CN_93314614_220000/RConn1 -- T_93314614_500000_ПС_Тагил/RConn1 -- _CN_93314614_220000_CN_96040535_220000/LConn1 -- L_93314614/LConn1
  _CN_275095874_220000_CN_93314614_220000/RConn2 -- T_93314614_500000_ПС_Тагил/RConn2 -- _CN_93314614_220000_CN_96040535_220000/LConn2 -- L_93314614/LConn2
  _CN_275095874_220000_CN_93314614_220000/RConn3 -- T_93314614_500000_ПС_Тагил/RConn3 -- _CN_93314614_220000_CN_96040535_220000/LConn3 -- L_93314614/LConn3 -- bus156/LConn1
  T_274851651_220000;110000_ПС_Первомайская/LConn1 -- ВЛ_220_кВ_Первомайская_–_Салда_CN_274851651_220000_CN_107585072_220000/LConn1
  T_274851651_220000;110000_ПС_Первомайская/LConn2 -- ВЛ_220_кВ_Первомайская_–_Салда_CN_274851651_220000_CN_107585072_220000/LConn2
  ВЛ_220_кВ_Первомайская_–_Салда_CN_274851651_220000_CN_107585072_220000/LConn3 -- T_274851651_220000;110000_ПС_Первомайская/LConn3 -- bus157/LConn1
  T_107585072_220000_ПС_Салда/LConn1 -- ВЛ_220_кВ_Первомайская_–_Салда_CN_274851651_220000_CN_107585072_220000/RConn1
  T_107585072_220000_ПС_Салда/LConn2 -- ВЛ_220_кВ_Первомайская_–_Салда_CN_274851651_220000_CN_107585072_220000/RConn2
  ВЛ_220_кВ_Первомайская_–_Салда_CN_274851651_220000_CN_107585072_220000/RConn3 -- T_107585072_220000_ПС_Салда/LConn3 -- bus158/LConn1
  _CN_209726497_220000_CN_239598452_220000/LConn1 -- T_209726497_220000_Подстанция_«Васильев»/LConn1 -- _CN_209726497_220000_CN_178844846_220000/LConn1
  _CN_209726497_220000_CN_239598452_220000/LConn2 -- T_209726497_220000_Подстанция_«Васильев»/LConn2 -- _CN_209726497_220000_CN_178844846_220000/LConn2
  _CN_209726497_220000_CN_239598452_220000/LConn3 -- T_209726497_220000_Подстанция_«Васильев»/LConn3 -- _CN_209726497_220000_CN_178844846_220000/LConn3 -- bus159/LConn1
  "T_239598452__Электроподстанция_220\\110\\35\"Кирьяновская\""/LConn1 -- _CN_209726497_220000_CN_239598452_220000/RConn1
  "T_239598452__Электроподстанция_220\\110\\35\"Кирьяновская\""/LConn2 -- _CN_209726497_220000_CN_239598452_220000/RConn2
  _CN_209726497_220000_CN_239598452_220000/RConn3 -- "T_239598452__Электроподстанция_220\\110\\35\"Кирьяновская\""/LConn3 -- bus160/LConn1
  T_178844846__/LConn1 -- _CN_209726497_220000_CN_178844846_220000/RConn1
  T_178844846__/LConn2 -- _CN_209726497_220000_CN_178844846_220000/RConn2
  _CN_209726497_220000_CN_178844846_220000/RConn3 -- T_178844846__/LConn3 -- bus161/LConn1
  _CN_130541748_220000_CN_68522408_220000/LConn1 -- T_130541748__/RConn1 -- L_130541748/LConn1
  _CN_130541748_220000_CN_68522408_220000/LConn2 -- T_130541748__/RConn2 -- L_130541748/LConn2
  _CN_130541748_220000_CN_68522408_220000/LConn3 -- T_130541748__/RConn3 -- L_130541748/LConn3 -- bus162/LConn1
  _CN_130541748_220000_CN_68522408_220000/RConn1 -- G_68522408_Нижневартовская_ГРЭС/RConn1 -- _CN_130541748_500000_CN_68522408_220000/LConn1 -- _CN_349543035_220000_CN_68522408_220000/LConn1 -- _CN_130503101_220000_CN_68522408_220000/LConn1 -- _CN_173759594_220000_CN_68522408_220000/LConn1
  _CN_130541748_220000_CN_68522408_220000/RConn2 -- G_68522408_Нижневартовская_ГРЭС/RConn2 -- _CN_130541748_500000_CN_68522408_220000/LConn2 -- _CN_349543035_220000_CN_68522408_220000/LConn2 -- _CN_130503101_220000_CN_68522408_220000/LConn2 -- _CN_173759594_220000_CN_68522408_220000/LConn2
  _CN_130541748_220000_CN_68522408_220000/RConn3 -- G_68522408_Нижневартовская_ГРЭС/RConn3 -- _CN_130541748_500000_CN_68522408_220000/LConn3 -- bus163/LConn1 -- _CN_349543035_220000_CN_68522408_220000/LConn3 -- _CN_130503101_220000_CN_68522408_220000/LConn3 -- _CN_173759594_220000_CN_68522408_220000/LConn3
  T_96040535_220000_ПС_Вязовская/LConn1 -- _CN_93314614_220000_CN_96040535_220000/RConn1
  T_96040535_220000_ПС_Вязовская/LConn2 -- _CN_93314614_220000_CN_96040535_220000/RConn2
  _CN_93314614_220000_CN_96040535_220000/RConn3 -- T_96040535_220000_ПС_Вязовская/LConn3 -- bus164/LConn1
  "T_349543035__ПС_\"Мираж\""/LConn1 -- _CN_349543035_220000_CN_68522408_220000/RConn1
  "T_349543035__ПС_\"Мираж\""/LConn2 -- _CN_349543035_220000_CN_68522408_220000/RConn2
  _CN_349543035_220000_CN_68522408_220000/RConn3 -- "T_349543035__ПС_\"Мираж\""/LConn3 -- bus165/LConn1
  T_96842811_110000_Карталы/LConn1 -- ВЛ_220_кВ_Троицкая_ГРЭС___Карталы_CN_96842811_220000_CN_109226934_220000/LConn1
  T_96842811_110000_Карталы/LConn2 -- ВЛ_220_кВ_Троицкая_ГРЭС___Карталы_CN_96842811_220000_CN_109226934_220000/LConn2
  ВЛ_220_кВ_Троицкая_ГРЭС___Карталы_CN_96842811_220000_CN_109226934_220000/LConn3 -- T_96842811_110000_Карталы/LConn3 -- bus166/LConn1
  ВЛ_220_кВ_Троицкая_ГРЭС___Карталы_CN_96842811_220000_CN_109226934_220000/RConn1 -- G_109226934_Троицкая_ГРЭС/RConn1 -- _CN_98423617_220000_CN_109226934_220000/LConn1 -- ВЛ_220кВ_Тр_ГРЭС_ПС90_1Л_CN_219112642_220000_CN_109226934_220000/LConn1 -- _CN_98423617_500000_CN_109226934_220000/LConn1 -- Тр_ГРЭС_Магнитогорск_CN_219112646_500000_CN_109226934_220000/LConn1
  ВЛ_220_кВ_Троицкая_ГРЭС___Карталы_CN_96842811_220000_CN_109226934_220000/RConn2 -- G_109226934_Троицкая_ГРЭС/RConn2 -- _CN_98423617_220000_CN_109226934_220000/LConn2 -- ВЛ_220кВ_Тр_ГРЭС_ПС90_1Л_CN_219112642_220000_CN_109226934_220000/LConn2 -- _CN_98423617_500000_CN_109226934_220000/LConn2 -- Тр_ГРЭС_Магнитогорск_CN_219112646_500000_CN_109226934_220000/LConn2
  ВЛ_220_кВ_Троицкая_ГРЭС___Карталы_CN_96842811_220000_CN_109226934_220000/RConn3 -- G_109226934_Троицкая_ГРЭС/RConn3 -- _CN_98423617_220000_CN_109226934_220000/LConn3 -- ВЛ_220кВ_Тр_ГРЭС_ПС90_1Л_CN_219112642_220000_CN_109226934_220000/LConn3 -- _CN_98423617_500000_CN_109226934_220000/LConn3 -- Тр_ГРЭС_Магнитогорск_CN_219112646_500000_CN_109226934_220000/LConn3 -- bus167/LConn1
  T_130503101_220000_Подстанция_«Советско_Соснинская»/LConn1 -- _CN_130503101_220000_CN_68522408_220000/RConn1
  T_130503101_220000_Подстанция_«Советско_Соснинская»/LConn2 -- _CN_130503101_220000_CN_68522408_220000/RConn2
  _CN_130503101_220000_CN_68522408_220000/RConn3 -- T_130503101_220000_Подстанция_«Советско_Соснинская»/LConn3 -- bus168/LConn1
  _CN_98423617_220000_CN_109226934_220000/RConn1 -- T_98423617_500000_Шагол/RConn1 -- _CN_98423617_220000_CN_86338059_220000/LConn1 -- _CN_98423617_220000_CN_106808187_220000/LConn1 -- _CN_98423617_220000_CN_102963612_220000/LConn1 -- _CN_98423617_220000_CN_166188874_220000/LConn1
  _CN_98423617_220000_CN_109226934_220000/RConn2 -- T_98423617_500000_Шагол/RConn2 -- _CN_98423617_220000_CN_86338059_220000/LConn2 -- _CN_98423617_220000_CN_106808187_220000/LConn2 -- _CN_98423617_220000_CN_102963612_220000/LConn2 -- _CN_98423617_220000_CN_166188874_220000/LConn2
  _CN_98423617_220000_CN_109226934_220000/RConn3 -- T_98423617_500000_Шагол/RConn3 -- _CN_98423617_220000_CN_86338059_220000/LConn3 -- _CN_98423617_220000_CN_106808187_220000/LConn3 -- bus169/LConn1 -- _CN_98423617_220000_CN_102963612_220000/LConn3 -- _CN_98423617_220000_CN_166188874_220000/LConn3
  G_102963612_Южноуральская_ГРЭС/RConn1 -- _CN_98423617_220000_CN_102963612_220000/RConn1
  G_102963612_Южноуральская_ГРЭС/RConn2 -- _CN_98423617_220000_CN_102963612_220000/RConn2
  _CN_98423617_220000_CN_102963612_220000/RConn3 -- G_102963612_Южноуральская_ГРЭС/RConn3 -- bus170/LConn1
  _CN_98423617_220000_CN_166188874_220000/RConn1 -- T_166188874_220000;110000;10000_Каменская/LConn1 -- _CN_93418566_220000_CN_166188874_220000/LConn1
  _CN_98423617_220000_CN_166188874_220000/RConn2 -- T_166188874_220000;110000;10000_Каменская/LConn2 -- _CN_93418566_220000_CN_166188874_220000/LConn2
  _CN_98423617_220000_CN_166188874_220000/RConn3 -- T_166188874_220000;110000;10000_Каменская/LConn3 -- _CN_93418566_220000_CN_166188874_220000/LConn3 -- bus171/LConn1
  T_86338059__/LConn1 -- _CN_98423617_220000_CN_86338059_220000/RConn1
  T_86338059__/LConn2 -- _CN_98423617_220000_CN_86338059_220000/RConn2
  _CN_98423617_220000_CN_86338059_220000/RConn3 -- T_86338059__/LConn3 -- bus172/LConn1
  T_106808187__/LConn1 -- _CN_98423617_220000_CN_106808187_220000/RConn1
  T_106808187__/LConn2 -- _CN_98423617_220000_CN_106808187_220000/RConn2
  _CN_98423617_220000_CN_106808187_220000/RConn3 -- T_106808187__/LConn3 -- bus173/LConn1
  T_219112642__ПС_90/LConn1 -- ВЛ_220кВ_Тр_ГРЭС_ПС90_1Л_CN_219112642_220000_CN_109226934_220000/RConn1
  T_219112642__ПС_90/LConn2 -- ВЛ_220кВ_Тр_ГРЭС_ПС90_1Л_CN_219112642_220000_CN_109226934_220000/RConn2
  ВЛ_220кВ_Тр_ГРЭС_ПС90_1Л_CN_219112642_220000_CN_109226934_220000/RConn3 -- T_219112642__ПС_90/LConn3 -- bus174/LConn1
  T_150165502_220000_ПС_Рябина/LConn1 -- _CN_81131204_220000_CN_150165502_220000/RConn1
  T_150165502_220000_ПС_Рябина/LConn2 -- _CN_81131204_220000_CN_150165502_220000/RConn2
  _CN_81131204_220000_CN_150165502_220000/RConn3 -- T_150165502_220000_ПС_Рябина/LConn3 -- bus175/LConn1
  T_93418566_220000;110000_Травянская/LConn1 -- _CN_93418566_220000_CN_166188874_220000/RConn1
  T_93418566_220000;110000_Травянская/LConn2 -- _CN_93418566_220000_CN_166188874_220000/RConn2
  _CN_93418566_220000_CN_166188874_220000/RConn3 -- T_93418566_220000;110000_Травянская/LConn3 -- bus176/LConn1
  T_300566433_220000;110000;10000_ПС_Белка/LConn1 -- ВЛ_220_кВ_ПС_БАЗ___ПС_Белка_CN_300566433_220000_CN_108718929_220000/LConn1
  T_300566433_220000;110000;10000_ПС_Белка/LConn2 -- ВЛ_220_кВ_ПС_БАЗ___ПС_Белка_CN_300566433_220000_CN_108718929_220000/LConn2
  ВЛ_220_кВ_ПС_БАЗ___ПС_Белка_CN_300566433_220000_CN_108718929_220000/LConn3 -- T_300566433_220000;110000;10000_ПС_Белка/LConn3 -- bus177/LConn1
  T_108718929_500000;220000;110000;10000_ПС_БАЗ/LConn1 -- ВЛ_220_кВ_ПС_БАЗ___ПС_Белка_CN_300566433_220000_CN_108718929_220000/RConn1
  T_108718929_500000;220000;110000;10000_ПС_БАЗ/LConn2 -- ВЛ_220_кВ_ПС_БАЗ___ПС_Белка_CN_300566433_220000_CN_108718929_220000/RConn2
  ВЛ_220_кВ_ПС_БАЗ___ПС_Белка_CN_300566433_220000_CN_108718929_220000/RConn3 -- T_108718929_500000;220000;110000;10000_ПС_БАЗ/LConn3 -- bus178/LConn1
  T_85603217__Сирень/LConn1 -- _CN_85603217_220000_CN_159955044_220000/LConn1
  T_85603217__Сирень/LConn2 -- _CN_85603217_220000_CN_159955044_220000/LConn2
  _CN_85603217_220000_CN_159955044_220000/LConn3 -- T_85603217__Сирень/LConn3 -- bus179/LConn1
  _CN_85603217_220000_CN_159955044_220000/RConn1 -- G_159955044_Рефтинская_ГРЭС/RConn1 -- _CN_93314614_500000_CN_159955044_220000/LConn1 -- _CN_117237579_500000_CN_159955044_220000/LConn1 -- _CN_27258925_500000_CN_159955044_220000/LConn1
  _CN_85603217_220000_CN_159955044_220000/RConn2 -- G_159955044_Рефтинская_ГРЭС/RConn2 -- _CN_93314614_500000_CN_159955044_220000/LConn2 -- _CN_117237579_500000_CN_159955044_220000/LConn2 -- _CN_27258925_500000_CN_159955044_220000/LConn2
  _CN_85603217_220000_CN_159955044_220000/RConn3 -- G_159955044_Рефтинская_ГРЭС/RConn3 -- _CN_93314614_500000_CN_159955044_220000/LConn3 -- _CN_117237579_500000_CN_159955044_220000/LConn3 -- bus180/LConn1 -- _CN_27258925_500000_CN_159955044_220000/LConn3
  T_173759594__Подстанция_Эмтор/LConn1 -- _CN_173759594_220000_CN_68522408_220000/RConn1
  T_173759594__Подстанция_Эмтор/LConn2 -- _CN_173759594_220000_CN_68522408_220000/RConn2
  _CN_173759594_220000_CN_68522408_220000/RConn3 -- T_173759594__Подстанция_Эмтор/LConn3 -- bus181/LConn1
  T_149575176__/LConn1 -- _CN_149575176_500000_CN_255065507_500000/LConn1
  T_149575176__/LConn2 -- _CN_149575176_500000_CN_255065507_500000/LConn2
  _CN_149575176_500000_CN_255065507_500000/LConn3 -- T_149575176__/LConn3 -- bus182/LConn1
  T_255065507_500000_Подстанция_«Тарко_Сале»/LConn1 -- _CN_149575176_500000_CN_255065507_500000/RConn1
  T_255065507_500000_Подстанция_«Тарко_Сале»/LConn2 -- _CN_149575176_500000_CN_255065507_500000/RConn2
  _CN_149575176_500000_CN_255065507_500000/RConn3 -- T_255065507_500000_Подстанция_«Тарко_Сале»/LConn3 -- bus183/LConn1
  _CN_145299338_500000_CN_27258925_500000/LConn1 -- "T_145299338__Электроподстанция_\"Нелым\""/LConn1 -- _CN_145299338_500000_CN_145299339_500000/LConn1
  _CN_145299338_500000_CN_27258925_500000/LConn2 -- "T_145299338__Электроподстанция_\"Нелым\""/LConn2 -- _CN_145299338_500000_CN_145299339_500000/LConn2
  _CN_145299338_500000_CN_27258925_500000/LConn3 -- "T_145299338__Электроподстанция_\"Нелым\""/LConn3 -- _CN_145299338_500000_CN_145299339_500000/LConn3 -- bus184/LConn1
  _CN_145299338_500000_CN_27258925_500000/RConn1 -- T_27258925_500000_ПС_Тюмень/LConn1 -- _CN_27258925_500000_CN_159955044_220000/RConn1 -- _CN_27258925_500000_CN_100289117_500000/LConn1
  _CN_145299338_500000_CN_27258925_500000/RConn2 -- T_27258925_500000_ПС_Тюмень/LConn2 -- _CN_27258925_500000_CN_159955044_220000/RConn2 -- _CN_27258925_500000_CN_100289117_500000/LConn2
  _CN_145299338_500000_CN_27258925_500000/RConn3 -- T_27258925_500000_ПС_Тюмень/LConn3 -- _CN_27258925_500000_CN_159955044_220000/RConn3 -- bus185/LConn1 -- _CN_27258925_500000_CN_100289117_500000/LConn3
  _CN_145299338_500000_CN_145299339_500000/RConn1 -- T_145299339__Электроподстанция/LConn1 -- _CN_145299339_500000_CN_100289117_500000/LConn1 -- _CN_145299339_500000_CN_121658984_500000/LConn1
  _CN_145299338_500000_CN_145299339_500000/RConn2 -- T_145299339__Электроподстанция/LConn2 -- _CN_145299339_500000_CN_100289117_500000/LConn2 -- _CN_145299339_500000_CN_121658984_500000/LConn2
  _CN_145299338_500000_CN_145299339_500000/RConn3 -- T_145299339__Электроподстанция/LConn3 -- _CN_145299339_500000_CN_100289117_500000/LConn3 -- _CN_145299339_500000_CN_121658984_500000/LConn3 -- bus186/LConn1
  _CN_145299339_500000_CN_100289117_500000/RConn1 -- T_100289117__/LConn1 -- _CN_27258925_500000_CN_100289117_500000/RConn1
  _CN_145299339_500000_CN_100289117_500000/RConn2 -- T_100289117__/LConn2 -- _CN_27258925_500000_CN_100289117_500000/RConn2
  _CN_145299339_500000_CN_100289117_500000/RConn3 -- T_100289117__/LConn3 -- _CN_27258925_500000_CN_100289117_500000/RConn3 -- bus187/LConn1
  G_121658984_ПС_500_кВ_Иртыш/RConn1 -- _CN_145299339_500000_CN_121658984_500000/RConn1
  G_121658984_ПС_500_кВ_Иртыш/RConn2 -- _CN_145299339_500000_CN_121658984_500000/RConn2
  _CN_145299339_500000_CN_121658984_500000/RConn3 -- G_121658984_ПС_500_кВ_Иртыш/RConn3 -- bus188/LConn1
  T_130506016_500000_Подстанция_«Сибирская»/LConn1 -- _CN_130506016_500000_CN_131369782_500000/LConn1
  T_130506016_500000_Подстанция_«Сибирская»/LConn2 -- _CN_130506016_500000_CN_131369782_500000/LConn2
  _CN_130506016_500000_CN_131369782_500000/LConn3 -- T_130506016_500000_Подстанция_«Сибирская»/LConn3 -- bus189/LConn1
  T_131369782_500000_Подстанция_«Трачуковская»/LConn1 -- _CN_130506016_500000_CN_131369782_500000/RConn1
  T_131369782_500000_Подстанция_«Трачуковская»/LConn2 -- _CN_130506016_500000_CN_131369782_500000/RConn2
  _CN_130506016_500000_CN_131369782_500000/RConn3 -- T_131369782_500000_Подстанция_«Трачуковская»/LConn3 -- bus190/LConn1
  _CN_100978216_500000_CN_41528780_500000/LConn1 -- T_100978216_500000_Челябинская/LConn1 -- _CN_100978216_500000_CN_98423617_500000/LConn1
  _CN_100978216_500000_CN_41528780_500000/LConn2 -- T_100978216_500000_Челябинская/LConn2 -- _CN_100978216_500000_CN_98423617_500000/LConn2
  _CN_100978216_500000_CN_41528780_500000/LConn3 -- T_100978216_500000_Челябинская/LConn3 -- _CN_100978216_500000_CN_98423617_500000/LConn3 -- bus191/LConn1
  _CN_100978216_500000_CN_41528780_500000/RConn1 -- T_41528780_500000_Подстанция_500_кВ___Златоуст/LConn1 -- _CN_41528780_500000_CN_169556579_500000/LConn1
  _CN_100978216_500000_CN_41528780_500000/RConn2 -- T_41528780_500000_Подстанция_500_кВ___Златоуст/LConn2 -- _CN_41528780_500000_CN_169556579_500000/LConn2
  _CN_100978216_500000_CN_41528780_500000/RConn3 -- T_41528780_500000_Подстанция_500_кВ___Златоуст/LConn3 -- _CN_41528780_500000_CN_169556579_500000/LConn3 -- bus192/LConn1
  _CN_100978216_500000_CN_98423617_500000/RConn1 -- T_98423617_500000_Шагол/LConn1 -- _CN_98423617_500000_CN_117237579_500000/LConn1 -- _CN_98423617_500000_CN_109226934_220000/RConn1
  _CN_100978216_500000_CN_98423617_500000/RConn2 -- T_98423617_500000_Шагол/LConn2 -- _CN_98423617_500000_CN_117237579_500000/LConn2 -- _CN_98423617_500000_CN_109226934_220000/RConn2
  _CN_100978216_500000_CN_98423617_500000/RConn3 -- T_98423617_500000_Шагол/LConn3 -- _CN_98423617_500000_CN_117237579_500000/LConn3 -- _CN_98423617_500000_CN_109226934_220000/RConn3 -- bus193/LConn1
  T_130541748__/LConn1 -- _CN_130541748_500000_CN_68522408_220000/RConn1
  T_130541748__/LConn2 -- _CN_130541748_500000_CN_68522408_220000/RConn2
  _CN_130541748_500000_CN_68522408_220000/RConn3 -- T_130541748__/LConn3 -- bus194/LConn1
  "T_99190583_500000;220000;110000;fixme_\"Смеловская\"_500_кВ"/LConn1 -- _CN_99190583_500000_CN_219112646_500000/LConn1
  "T_99190583_500000;220000;110000;fixme_\"Смеловская\"_500_кВ"/LConn2 -- _CN_99190583_500000_CN_219112646_500000/LConn2
  _CN_99190583_500000_CN_219112646_500000/LConn3 -- "T_99190583_500000;220000;110000;fixme_\"Смеловская\"_500_кВ"/LConn3 -- bus195/LConn1
  _CN_99190583_500000_CN_219112646_500000/RConn1 -- T_219112646__/LConn1 -- Тр_ГРЭС_Магнитогорск_CN_219112646_500000_CN_109226934_220000/RConn1
  _CN_99190583_500000_CN_219112646_500000/RConn2 -- T_219112646__/LConn2 -- Тр_ГРЭС_Магнитогорск_CN_219112646_500000_CN_109226934_220000/RConn2
  _CN_99190583_500000_CN_219112646_500000/RConn3 -- T_219112646__/LConn3 -- Тр_ГРЭС_Магнитогорск_CN_219112646_500000_CN_109226934_220000/RConn3 -- bus196/LConn1
  _CN_98423617_500000_CN_117237579_500000/RConn1 -- T_117237579__/LConn1 -- _CN_117237579_500000_CN_159955044_220000/RConn1
  _CN_98423617_500000_CN_117237579_500000/RConn2 -- T_117237579__/LConn2 -- _CN_117237579_500000_CN_159955044_220000/RConn2
  _CN_98423617_500000_CN_117237579_500000/RConn3 -- T_117237579__/LConn3 -- _CN_117237579_500000_CN_159955044_220000/RConn3 -- bus197/LConn1
  T_93314614_500000_ПС_Тагил/LConn1 -- _CN_93314614_500000_CN_159955044_220000/RConn1
  T_93314614_500000_ПС_Тагил/LConn2 -- _CN_93314614_500000_CN_159955044_220000/RConn2
  _CN_93314614_500000_CN_159955044_220000/RConn3 -- T_93314614_500000_ПС_Тагил/LConn3 -- bus198/LConn1
  _CN_41528780_500000_CN_169556579_500000/RConn1 -- T_169556579__ПC_Приваловская_500_кВ/LConn1 -- ВЛ_500кВ_Кропачево___Приваловская_CN_169556579_500000_CN_113767652_500000/LConn1
  _CN_41528780_500000_CN_169556579_500000/RConn2 -- T_169556579__ПC_Приваловская_500_кВ/LConn2 -- ВЛ_500кВ_Кропачево___Приваловская_CN_169556579_500000_CN_113767652_500000/LConn2
  _CN_41528780_500000_CN_169556579_500000/RConn3 -- T_169556579__ПC_Приваловская_500_кВ/LConn3 -- ВЛ_500кВ_Кропачево___Приваловская_CN_169556579_500000_CN_113767652_500000/LConn3 -- bus199/LConn1
  T_244062688_500000_Подстанция_«Ильково»/LConn1 -- _CN_244062688_500000_CN_163913701_500000/LConn1
  T_244062688_500000_Подстанция_«Ильково»/LConn2 -- _CN_244062688_500000_CN_163913701_500000/LConn2
  _CN_244062688_500000_CN_163913701_500000/LConn3 -- T_244062688_500000_Подстанция_«Ильково»/LConn3 -- bus200/LConn1
  T_163913701__/LConn1 -- _CN_244062688_500000_CN_163913701_500000/RConn1
  T_163913701__/LConn2 -- _CN_244062688_500000_CN_163913701_500000/RConn2
  _CN_244062688_500000_CN_163913701_500000/RConn3 -- T_163913701__/LConn3 -- bus201/LConn1
  T_113767652_500000_ПС_Кропачево/LConn1 -- ВЛ_500кВ_Кропачево___Приваловская_CN_169556579_500000_CN_113767652_500000/RConn1
  T_113767652_500000_ПС_Кропачево/LConn2 -- ВЛ_500кВ_Кропачево___Приваловская_CN_169556579_500000_CN_113767652_500000/RConn2
  ВЛ_500кВ_Кропачево___Приваловская_CN_169556579_500000_CN_113767652_500000/RConn3 -- T_113767652_500000_ПС_Кропачево/LConn3 -- bus202/LConn1
  T_218733056__/RConn1 -- L_218733056/LConn1
  T_218733056__/RConn2 -- L_218733056/LConn2
  L_218733056/LConn3 -- T_218733056__/RConn3 -- bus203/LConn1
  T_218733818__/RConn1 -- L_218733818/LConn1
  T_218733818__/RConn2 -- L_218733818/LConn2
  L_218733818/LConn3 -- T_218733818__/RConn3 -- bus204/LConn1
  T_218733820__/RConn1 -- L_218733820/LConn1
  T_218733820__/RConn2 -- L_218733820/LConn2
  L_218733820/LConn3 -- T_218733820__/RConn3 -- bus205/LConn1
  T_128448427__/RConn1 -- L_128448427/LConn1
  T_128448427__/RConn2 -- L_128448427/LConn2
  L_128448427/LConn3 -- T_128448427__/RConn3 -- bus206/LConn1
  T_40080294_110000;10000_Московская/RConn1 -- L_40080294/LConn1
  T_40080294_110000;10000_Московская/RConn2 -- L_40080294/LConn2
  L_40080294/LConn3 -- T_40080294_110000;10000_Московская/RConn3 -- bus207/LConn1
  T_310639917_110000;10000_Отрадная/RConn1 -- L_310639917/LConn1
  T_310639917_110000;10000_Отрадная/RConn2 -- L_310639917/LConn2
  L_310639917/LConn3 -- T_310639917_110000;10000_Отрадная/RConn3 -- bus208/LConn1
  T_78488044__Академическая/RConn1 -- L_78488044/LConn1
  T_78488044__Академическая/RConn2 -- L_78488044/LConn2
  L_78488044/LConn3 -- T_78488044__Академическая/RConn3 -- bus209/LConn1
  T_97827873__Овощная/RConn1 -- L_97827873/LConn1
  T_97827873__Овощная/RConn2 -- L_97827873/LConn2
  L_97827873/LConn3 -- T_97827873__Овощная/RConn3 -- bus210/LConn1
  T_42918338__Ясная/RConn1 -- L_42918338/LConn1
  T_42918338__Ясная/RConn2 -- L_42918338/LConn2
  L_42918338/LConn3 -- T_42918338__Ясная/RConn3 -- bus211/LConn1
  T_331102892__Бараба/RConn1 -- L_331102892/LConn1
  T_331102892__Бараба/RConn2 -- L_331102892/LConn2
  L_331102892/LConn3 -- T_331102892__Бараба/RConn3 -- bus212/LConn1
  T_128346488__Грязновская/RConn1 -- L_128346488/LConn1
  T_128346488__Грязновская/RConn2 -- L_128346488/LConn2
  L_128346488/LConn3 -- T_128346488__Грязновская/RConn3 -- bus213/LConn1
  T_164371995__/RConn1 -- L_164371995/LConn1
  T_164371995__/RConn2 -- L_164371995/LConn2
  L_164371995/LConn3 -- T_164371995__/RConn3 -- bus214/LConn1
  T_187971431__Клевакино/RConn1 -- L_187971431/LConn1
  T_187971431__Клевакино/RConn2 -- L_187971431/LConn2
  L_187971431/LConn3 -- T_187971431__Клевакино/RConn3 -- bus215/LConn1
  T_93050981__Черемхово/RConn1 -- L_93050981/LConn1
  T_93050981__Черемхово/RConn2 -- L_93050981/LConn2
  L_93050981/LConn3 -- T_93050981__Черемхово/RConn3 -- bus216/LConn1
  T_320347053__Кочневское/RConn1 -- L_320347053/LConn1
  T_320347053__Кочневское/RConn2 -- L_320347053/LConn2
  L_320347053/LConn3 -- T_320347053__Кочневское/RConn3 -- bus217/LConn1
  T_279497233__/RConn1 -- L_279497233/LConn1
  T_279497233__/RConn2 -- L_279497233/LConn2
  L_279497233/LConn3 -- T_279497233__/RConn3 -- bus218/LConn1
  T_126093674__/RConn1 -- L_126093674/LConn1
  T_126093674__/RConn2 -- L_126093674/LConn2
  L_126093674/LConn3 -- T_126093674__/RConn3 -- bus219/LConn1
  "T_96989715_110000;6000_ПС_\"Кварц\""/RConn1 -- L_96989715/LConn1
  "T_96989715_110000;6000_ПС_\"Кварц\""/RConn2 -- L_96989715/LConn2
  L_96989715/LConn3 -- "T_96989715_110000;6000_ПС_\"Кварц\""/RConn3 -- bus220/LConn1
  T_93260139__Родник/RConn1 -- L_93260139/LConn1
  T_93260139__Родник/RConn2 -- L_93260139/LConn2
  L_93260139/LConn3 -- T_93260139__Родник/RConn3 -- bus221/LConn1
  "T_274652249__П_ст_110_35_6кВ_\"Атиг\""/RConn1 -- L_274652249/LConn1
  "T_274652249__П_ст_110_35_6кВ_\"Атиг\""/RConn2 -- L_274652249/LConn2
  L_274652249/LConn3 -- "T_274652249__П_ст_110_35_6кВ_\"Атиг\""/RConn3 -- bus222/LConn1
  "T_216208030_110000;35000;6000_ПС_\"Бисерть\""/RConn1 -- L_216208030/LConn1
  "T_216208030_110000;35000;6000_ПС_\"Бисерть\""/RConn2 -- L_216208030/LConn2
  L_216208030/LConn3 -- "T_216208030_110000;35000;6000_ПС_\"Бисерть\""/RConn3 -- bus223/LConn1
  T_106927870__/RConn1 -- L_106927870/LConn1
  T_106927870__/RConn2 -- L_106927870/LConn2
  L_106927870/LConn3 -- T_106927870__/RConn3 -- bus224/LConn1
  T_255624915__/RConn1 -- L_255624915/LConn1
  T_255624915__/RConn2 -- L_255624915/LConn2
  L_255624915/LConn3 -- T_255624915__/RConn3 -- bus225/LConn1
  T_153740317_110000_ГОРНЫЙ_ЩИТ/RConn1 -- L_153740317/LConn1
  T_153740317_110000_ГОРНЫЙ_ЩИТ/RConn2 -- L_153740317/LConn2
  L_153740317/LConn3 -- T_153740317_110000_ГОРНЫЙ_ЩИТ/RConn3 -- bus226/LConn1
  T_153741014__/RConn1 -- L_153741014/LConn1
  T_153741014__/RConn2 -- L_153741014/LConn2
  L_153741014/LConn3 -- T_153741014__/RConn3 -- bus227/LConn1
  T_282779585__/RConn1 -- L_282779585/LConn1
  T_282779585__/RConn2 -- L_282779585/LConn2
  L_282779585/LConn3 -- T_282779585__/RConn3 -- bus228/LConn1
  T_282779587__/RConn1 -- L_282779587/LConn1
  T_282779587__/RConn2 -- L_282779587/LConn2
  L_282779587/LConn3 -- T_282779587__/RConn3 -- bus229/LConn1
  T_282645278__/RConn1 -- L_282645278/LConn1
  T_282645278__/RConn2 -- L_282645278/LConn2
  L_282645278/LConn3 -- T_282645278__/RConn3 -- bus230/LConn1
  T_121211432__Ильменская/RConn1 -- L_121211432/LConn1
  T_121211432__Ильменская/RConn2 -- L_121211432/LConn2
  L_121211432/LConn3 -- T_121211432__Ильменская/RConn3 -- bus231/LConn1
  T_372580506_110000_Кулуево/RConn1 -- L_372580506/LConn1
  T_372580506_110000_Кулуево/RConn2 -- L_372580506/LConn2
  L_372580506/LConn3 -- T_372580506_110000_Кулуево/RConn3 -- bus232/LConn1
  T_372580526_110000_Яраткулова/RConn1 -- L_372580526/LConn1
  T_372580526_110000_Яраткулова/RConn2 -- L_372580526/LConn2
  L_372580526/LConn3 -- T_372580526_110000_Яраткулова/RConn3 -- bus233/LConn1
  T_116299140_110000_Чебаркуль/RConn1 -- L_116299140/LConn1
  T_116299140_110000_Чебаркуль/RConn2 -- L_116299140/LConn2
  L_116299140/LConn3 -- T_116299140_110000_Чебаркуль/RConn3 -- bus234/LConn1
  T_189890975_110000_Тургояк/RConn1 -- L_189890975/LConn1
  T_189890975_110000_Тургояк/RConn2 -- L_189890975/LConn2
  L_189890975/LConn3 -- T_189890975_110000_Тургояк/RConn3 -- bus235/LConn1
  "T_115954225__ПС_\"Сухоборка\"_110_10"/RConn1 -- L_115954225/LConn1
  "T_115954225__ПС_\"Сухоборка\"_110_10"/RConn2 -- L_115954225/LConn2
  L_115954225/LConn3 -- "T_115954225__ПС_\"Сухоборка\"_110_10"/RConn3 -- bus236/LConn1
  "T_115981920__ПС_\"Щучье_тяга\"_110_10"/RConn1 -- L_115981920/LConn1
  "T_115981920__ПС_\"Щучье_тяга\"_110_10"/RConn2 -- L_115981920/LConn2
  L_115981920/LConn3 -- "T_115981920__ПС_\"Щучье_тяга\"_110_10"/RConn3 -- bus237/LConn1
  "T_115951342__ПС_\"Нифанка\"_110_10"/RConn1 -- L_115951342/LConn1
  "T_115951342__ПС_\"Нифанка\"_110_10"/RConn2 -- L_115951342/LConn2
  L_115951342/LConn3 -- "T_115951342__ПС_\"Нифанка\"_110_10"/RConn3 -- bus238/LConn1
  "T_117325674__ПС_\"Сафакулево\"_110_10"/RConn1 -- L_117325674/LConn1
  "T_117325674__ПС_\"Сафакулево\"_110_10"/RConn2 -- L_117325674/LConn2
  L_117325674/LConn3 -- "T_117325674__ПС_\"Сафакулево\"_110_10"/RConn3 -- bus239/LConn1
  T_144702516__/RConn1 -- L_144702516/LConn1
  T_144702516__/RConn2 -- L_144702516/LConn2
  L_144702516/LConn3 -- T_144702516__/RConn3 -- bus240/LConn1
  T_163401683_110000_Бреды/RConn1 -- L_163401683/LConn1
  T_163401683_110000_Бреды/RConn2 -- L_163401683/LConn2
  L_163401683/LConn3 -- T_163401683_110000_Бреды/RConn3 -- bus241/LConn1
  T_286951577_110000_/RConn1 -- L_286951577/LConn1
  T_286951577_110000_/RConn2 -- L_286951577/LConn2
  L_286951577/LConn3 -- T_286951577_110000_/RConn3 -- bus242/LConn1
  T_254457038_110000_Аненская/RConn1 -- L_254457038/LConn1
  T_254457038_110000_Аненская/RConn2 -- L_254457038/LConn2
  L_254457038/LConn3 -- T_254457038_110000_Аненская/RConn3 -- bus243/LConn1
  T_351136526_110000_/RConn1 -- L_351136526/LConn1
  T_351136526_110000_/RConn2 -- L_351136526/LConn2
  L_351136526/LConn3 -- T_351136526_110000_/RConn3 -- bus244/LConn1
  T_280421437__/RConn1 -- L_280421437/LConn1
  T_280421437__/RConn2 -- L_280421437/LConn2
  L_280421437/LConn3 -- T_280421437__/RConn3 -- bus245/LConn1
  T_275095838_110000;10000_Школьная/RConn1 -- L_275095838/LConn1
  T_275095838_110000;10000_Школьная/RConn2 -- L_275095838/LConn2
  L_275095838/LConn3 -- T_275095838_110000;10000_Школьная/RConn3 -- bus246/LConn1
  T_37479179__УЗХР/RConn1 -- L_37479179/LConn1
  T_37479179__УЗХР/RConn2 -- L_37479179/LConn2
  L_37479179/LConn3 -- T_37479179__УЗХР/RConn3 -- bus247/LConn1
  T_76449471_110000;10000_ПС_«Веер»/RConn1 -- L_76449471/LConn1
  T_76449471_110000;10000_ПС_«Веер»/RConn2 -- L_76449471/LConn2
  L_76449471/LConn3 -- T_76449471_110000;10000_ПС_«Веер»/RConn3 -- bus248/LConn1
  T_66264428__Среднеуральская/RConn1 -- L_66264428/LConn1
  T_66264428__Среднеуральская/RConn2 -- L_66264428/LConn2
  L_66264428/LConn3 -- T_66264428__Среднеуральская/RConn3 -- bus249/LConn1
  T_131114928__Термическая/RConn1 -- L_131114928/LConn1
  T_131114928__Термическая/RConn2 -- L_131114928/LConn2
  L_131114928/LConn3 -- T_131114928__Термическая/RConn3 -- bus250/LConn1
  T_317157140_110000;6000_ПС_Электромедь/RConn1 -- L_317157140/LConn1
  T_317157140_110000;6000_ПС_Электромедь/RConn2 -- L_317157140/LConn2
  L_317157140/LConn3 -- T_317157140_110000;6000_ПС_Электромедь/RConn3 -- bus251/LConn1
  T_276394749_110000;6000_ПС_Рудянка/RConn1 -- L_276394749/LConn1
  T_276394749_110000;6000_ПС_Рудянка/RConn2 -- L_276394749/LConn2
  L_276394749/LConn3 -- T_276394749_110000;6000_ПС_Рудянка/RConn3 -- bus252/LConn1
  T_273707087__ГПП_«Солнечная»/RConn1 -- L_273707087/LConn1
  T_273707087__ГПП_«Солнечная»/RConn2 -- L_273707087/LConn2
  L_273707087/LConn3 -- T_273707087__ГПП_«Солнечная»/RConn3 -- bus253/LConn1
  T_110538007_220000;110000;35000_ПС_«Окунево»/RConn1 -- L_110538007/LConn1
  T_110538007_220000;110000;35000_ПС_«Окунево»/RConn2 -- L_110538007/LConn2
  L_110538007/LConn3 -- T_110538007_220000;110000;35000_ПС_«Окунево»/RConn3 -- bus254/LConn1
  T_250194000__ПС_Арси/RConn1 -- L_250194000/LConn1
  T_250194000__ПС_Арси/RConn2 -- L_250194000/LConn2
  L_250194000/LConn3 -- T_250194000__ПС_Арси/RConn3 -- bus255/LConn1
  T_191446930__Подстанция/RConn1 -- L_191446930/LConn1
  T_191446930__Подстанция/RConn2 -- L_191446930/LConn2
  L_191446930/LConn3 -- T_191446930__Подстанция/RConn3 -- bus256/LConn1
  T_139662419_110000_/RConn1 -- L_139662419/LConn1
  T_139662419_110000_/RConn2 -- L_139662419/LConn2
  L_139662419/LConn3 -- T_139662419_110000_/RConn3 -- bus257/LConn1
  T_165574395_110000_Таганай/RConn1 -- L_165574395/LConn1
  T_165574395_110000_Таганай/RConn2 -- L_165574395/LConn2
  L_165574395/LConn3 -- T_165574395_110000_Таганай/RConn3 -- bus258/LConn1
  T_26354372_110000_Миасс/RConn1 -- L_26354372/LConn1
  T_26354372_110000_Миасс/RConn2 -- L_26354372/LConn2
  L_26354372/LConn3 -- T_26354372_110000_Миасс/RConn3 -- bus259/LConn1
  T_99731541__/RConn1 -- L_99731541/LConn1
  T_99731541__/RConn2 -- L_99731541/LConn2
  L_99731541/LConn3 -- T_99731541__/RConn3 -- bus260/LConn1
  T_101747976__/RConn1 -- L_101747976/LConn1
  T_101747976__/RConn2 -- L_101747976/LConn2
  L_101747976/LConn3 -- T_101747976__/RConn3 -- bus261/LConn1
  T_99875927__/RConn1 -- L_99875927/LConn1
  T_99875927__/RConn2 -- L_99875927/LConn2
  L_99875927/LConn3 -- T_99875927__/RConn3 -- bus262/LConn1
  T_101594027__/RConn1 -- L_101594027/LConn1
  T_101594027__/RConn2 -- L_101594027/LConn2
  L_101594027/LConn3 -- T_101594027__/RConn3 -- bus263/LConn1
  T_99869836__Бульварная/RConn1 -- L_99869836/LConn1
  T_99869836__Бульварная/RConn2 -- L_99869836/LConn2
  L_99869836/LConn3 -- T_99869836__Бульварная/RConn3 -- bus264/LConn1
  T_361266572_110000_Гранит/RConn1 -- L_361266572/LConn1
  T_361266572_110000_Гранит/RConn2 -- L_361266572/LConn2
  L_361266572/LConn3 -- T_361266572_110000_Гранит/RConn3 -- bus265/LConn1
  T_117325672__ПС_Пивкино_Тяга_110_10/RConn1 -- L_117325672/LConn1
  T_117325672__ПС_Пивкино_Тяга_110_10/RConn2 -- L_117325672/LConn2
  L_117325672/LConn3 -- T_117325672__ПС_Пивкино_Тяга_110_10/RConn3 -- bus266/LConn1
  T_117325678__ПС_Алакуль_Тяга_110_10/RConn1 -- L_117325678/LConn1
  T_117325678__ПС_Алакуль_Тяга_110_10/RConn2 -- L_117325678/LConn2
  L_117325678/LConn3 -- T_117325678__ПС_Алакуль_Тяга_110_10/RConn3 -- bus267/LConn1
  T_106889826__/RConn1 -- L_106889826/LConn1
  T_106889826__/RConn2 -- L_106889826/LConn2
  L_106889826/LConn3 -- T_106889826__/RConn3 -- bus268/LConn1
  T_235846243_110000;6000_ПС_Першино/RConn1 -- L_235846243/LConn1
  T_235846243_110000;6000_ПС_Першино/RConn2 -- L_235846243/LConn2
  L_235846243/LConn3 -- T_235846243_110000;6000_ПС_Першино/RConn3 -- bus269/LConn1
  T_281707739_110000;35000;6000_ПС_Черёмухово/RConn1 -- L_281707739/LConn1
  T_281707739_110000;35000;6000_ПС_Черёмухово/RConn2 -- L_281707739/LConn2
  L_281707739/LConn3 -- T_281707739_110000;35000;6000_ПС_Черёмухово/RConn3 -- bus270/LConn1
  T_182904423__/RConn1 -- L_182904423/LConn1
  T_182904423__/RConn2 -- L_182904423/LConn2
  L_182904423/LConn3 -- T_182904423__/RConn3 -- bus271/LConn1
  T_230206278__/RConn1 -- L_230206278/LConn1
  T_230206278__/RConn2 -- L_230206278/LConn2
  L_230206278/LConn3 -- T_230206278__/RConn3 -- bus272/LConn1
  T_225283934__Электроподстанция/RConn1 -- L_225283934/LConn1
  T_225283934__Электроподстанция/RConn2 -- L_225283934/LConn2
  L_225283934/LConn3 -- T_225283934__Электроподстанция/RConn3 -- bus273/LConn1
  T_200241256_110000;10000_ПС_Яр/RConn1 -- L_200241256/LConn1
  T_200241256_110000;10000_ПС_Яр/RConn2 -- L_200241256/LConn2
  L_200241256/LConn3 -- T_200241256_110000;10000_ПС_Яр/RConn3 -- bus274/LConn1
  T_279664560_110000;10000_ПС_Юшала/RConn1 -- L_279664560/LConn1
  T_279664560_110000;10000_ПС_Юшала/RConn2 -- L_279664560/LConn2
  L_279664560/LConn3 -- T_279664560_110000;10000_ПС_Юшала/RConn3 -- bus275/LConn1
  T_280145603_110000;10000_ПС_Истоур/RConn1 -- L_280145603/LConn1
  T_280145603_110000;10000_ПС_Истоур/RConn2 -- L_280145603/LConn2
  L_280145603/LConn3 -- T_280145603_110000;10000_ПС_Истоур/RConn3 -- bus276/LConn1
  T_114780778__Новоградская/RConn1 -- L_114780778/LConn1
  T_114780778__Новоградская/RConn2 -- L_114780778/LConn2
  L_114780778/LConn3 -- T_114780778__Новоградская/RConn3 -- bus277/LConn1
  T_100306689__Спортивная/RConn1 -- L_100306689/LConn1
  T_100306689__Спортивная/RConn2 -- L_100306689/LConn2
  L_100306689/LConn3 -- T_100306689__Спортивная/RConn3 -- bus278/LConn1
  T_199389117__Подстанция/RConn1 -- L_199389117/LConn1
  T_199389117__Подстанция/RConn2 -- L_199389117/LConn2
  L_199389117/LConn3 -- T_199389117__Подстанция/RConn3 -- bus279/LConn1
  T_339193644__/RConn1 -- L_339193644/LConn1
  T_339193644__/RConn2 -- L_339193644/LConn2
  L_339193644/LConn3 -- T_339193644__/RConn3 -- bus280/LConn1
  T_118008950__/RConn1 -- L_118008950/LConn1
  T_118008950__/RConn2 -- L_118008950/LConn2
  L_118008950/LConn3 -- T_118008950__/RConn3 -- bus281/LConn1
  T_117941010__ПС_Чудиново_110_10/RConn1 -- L_117941010/LConn1
  T_117941010__ПС_Чудиново_110_10/RConn2 -- L_117941010/LConn2
  L_117941010/LConn3 -- T_117941010__ПС_Чудиново_110_10/RConn3 -- bus282/LConn1
  T_144437268__Автозаводская/RConn1 -- L_144437268/LConn1
  T_144437268__Автозаводская/RConn2 -- L_144437268/LConn2
  L_144437268/LConn3 -- T_144437268__Автозаводская/RConn3 -- bus283/LConn1
  T_273461546_110000;10000_ПС_Киприно/RConn1 -- L_273461546/LConn1
  T_273461546_110000;10000_ПС_Киприно/RConn2 -- L_273461546/LConn2
  L_273461546/LConn3 -- T_273461546_110000;10000_ПС_Киприно/RConn3 -- bus284/LConn1
  T_273649961_110000;35000;10000_ПС_Черемисска/RConn1 -- L_273649961/LConn1
  T_273649961_110000;35000;10000_ПС_Черемисска/RConn2 -- L_273649961/LConn2
  L_273649961/LConn3 -- T_273649961_110000;35000;10000_ПС_Черемисска/RConn3 -- bus285/LConn1
  T_101532642_110000;35000;10000_ПС_Таволги/RConn1 -- L_101532642/LConn1
  T_101532642_110000;35000;10000_ПС_Таволги/RConn2 -- L_101532642/LConn2
  L_101532642/LConn3 -- T_101532642_110000;35000;10000_ПС_Таволги/RConn3 -- bus286/LConn1
  T_135780398__/RConn1 -- L_135780398/LConn1
  T_135780398__/RConn2 -- L_135780398/LConn2
  L_135780398/LConn3 -- T_135780398__/RConn3 -- bus287/LConn1
  T_306102396__/RConn1 -- L_306102396/LConn1
  T_306102396__/RConn2 -- L_306102396/LConn2
  L_306102396/LConn3 -- T_306102396__/RConn3 -- bus288/LConn1
  T_305096727__/RConn1 -- L_305096727/LConn1
  T_305096727__/RConn2 -- L_305096727/LConn2
  L_305096727/LConn3 -- T_305096727__/RConn3 -- bus289/LConn1
  T_117941027__ПС_Сулейманово_110_35_10/RConn1 -- L_117941027/LConn1
  T_117941027__ПС_Сулейманово_110_35_10/RConn2 -- L_117941027/LConn2
  L_117941027/LConn3 -- T_117941027__ПС_Сулейманово_110_35_10/RConn3 -- bus290/LConn1
  T_104952455__ПС_Уфалей/RConn1 -- L_104952455/LConn1
  T_104952455__ПС_Уфалей/RConn2 -- L_104952455/LConn2
  L_104952455/LConn3 -- T_104952455__ПС_Уфалей/RConn3 -- bus291/LConn1
  T_196250439__/RConn1 -- L_196250439/LConn1
  T_196250439__/RConn2 -- L_196250439/LConn2
  L_196250439/LConn3 -- T_196250439__/RConn3 -- bus292/LConn1
  T_361265069_110000_Мисяш/RConn1 -- L_361265069/LConn1
  T_361265069_110000_Мисяш/RConn2 -- L_361265069/LConn2
  L_361265069/LConn3 -- T_361265069_110000_Мисяш/RConn3 -- bus293/LConn1
  T_266070665__Измоденово/RConn1 -- L_266070665/LConn1
  T_266070665__Измоденово/RConn2 -- L_266070665/LConn2
  L_266070665/LConn3 -- T_266070665__Измоденово/RConn3 -- bus294/LConn1
  T_130127057__/RConn1 -- L_130127057/LConn1
  T_130127057__/RConn2 -- L_130127057/LConn2
  L_130127057/LConn3 -- T_130127057__/RConn3 -- bus295/LConn1
  T_139658378__/RConn1 -- L_139658378/LConn1
  T_139658378__/RConn2 -- L_139658378/LConn2
  L_139658378/LConn3 -- T_139658378__/RConn3 -- bus296/LConn1
  T_139658358__Северная/RConn1 -- L_139658358/LConn1
  T_139658358__Северная/RConn2 -- L_139658358/LConn2
  L_139658358/LConn3 -- T_139658358__Северная/RConn3 -- bus297/LConn1
  T_354777580__/RConn1 -- L_354777580/LConn1
  T_354777580__/RConn2 -- L_354777580/LConn2
  L_354777580/LConn3 -- T_354777580__/RConn3 -- bus298/LConn1
  T_168166544_110000;fixme_/RConn1 -- L_168166544/LConn1
  T_168166544_110000;fixme_/RConn2 -- L_168166544/LConn2
  L_168166544/LConn3 -- T_168166544_110000;fixme_/RConn3 -- bus299/LConn1
  T_168174311__/RConn1 -- L_168174311/LConn1
  T_168174311__/RConn2 -- L_168174311/LConn2
  L_168174311/LConn3 -- T_168174311__/RConn3 -- bus300/LConn1
  T_105584274_110000;6000_ПС_Черноисточинск/RConn1 -- L_105584274/LConn1
  T_105584274_110000;6000_ПС_Черноисточинск/RConn2 -- L_105584274/LConn2
  L_105584274/LConn3 -- T_105584274_110000;6000_ПС_Черноисточинск/RConn3 -- bus301/LConn1
  T_274851642_110000;6000_ПС_НЦЗ/RConn1 -- L_274851642/LConn1
  T_274851642_110000;6000_ПС_НЦЗ/RConn2 -- L_274851642/LConn2
  L_274851642/LConn3 -- T_274851642_110000;6000_ПС_НЦЗ/RConn3 -- bus302/LConn1
  T_361264295_110000_Луговая/RConn1 -- L_361264295/LConn1
  T_361264295_110000_Луговая/RConn2 -- L_361264295/LConn2
  L_361264295/LConn3 -- T_361264295_110000_Луговая/RConn3 -- bus303/LConn1
  T_372580522_110000_Тимирязевская/RConn1 -- L_372580522/LConn1
  T_372580522_110000_Тимирязевская/RConn2 -- L_372580522/LConn2
  L_372580522/LConn3 -- T_372580522_110000_Тимирязевская/RConn3 -- bus304/LConn1
  T_97947939__ПС_«Загородная»/RConn1 -- L_97947939/LConn1
  T_97947939__ПС_«Загородная»/RConn2 -- L_97947939/LConn2
  L_97947939/LConn3 -- T_97947939__ПС_«Загородная»/RConn3 -- bus305/LConn1
  T_176374151__Унипромедь/RConn1 -- L_176374151/LConn1
  T_176374151__Унипромедь/RConn2 -- L_176374151/LConn2
  L_176374151/LConn3 -- T_176374151__Унипромедь/RConn3 -- bus306/LConn1
  T_38919677__Сибирская/RConn1 -- L_38919677/LConn1
  T_38919677__Сибирская/RConn2 -- L_38919677/LConn2
  L_38919677/LConn3 -- T_38919677__Сибирская/RConn3 -- bus307/LConn1
  T_352282301_110000_Тумак/RConn1 -- L_352282301/LConn1
  T_352282301_110000_Тумак/RConn2 -- L_352282301/LConn2
  L_352282301/LConn3 -- T_352282301_110000_Тумак/RConn3 -- bus308/LConn1
  T_138410290_110000_Варна/RConn1 -- L_138410290/LConn1
  T_138410290_110000_Варна/RConn2 -- L_138410290/LConn2
  L_138410290/LConn3 -- T_138410290_110000_Варна/RConn3 -- bus309/LConn1
  T_190450368_110000_Подстанция_«Григорьевская»/RConn1 -- L_190450368/LConn1
  T_190450368_110000_Подстанция_«Григорьевская»/RConn2 -- L_190450368/LConn2
  L_190450368/LConn3 -- T_190450368_110000_Подстанция_«Григорьевская»/RConn3 -- bus310/LConn1
  T_89555905_110000_Подстанция_«Стрежевская»/RConn1 -- L_89555905/LConn1
  T_89555905_110000_Подстанция_«Стрежевская»/RConn2 -- L_89555905/LConn2
  L_89555905/LConn3 -- T_89555905_110000_Подстанция_«Стрежевская»/RConn3 -- bus311/LConn1
  T_325873379__/RConn1 -- L_325873379/LConn1
  T_325873379__/RConn2 -- L_325873379/LConn2
  L_325873379/LConn3 -- T_325873379__/RConn3 -- bus312/LConn1
  T_90797306__/RConn1 -- L_90797306/LConn1
  T_90797306__/RConn2 -- L_90797306/LConn2
  L_90797306/LConn3 -- T_90797306__/RConn3 -- bus313/LConn1
  T_130534123__/RConn1 -- L_130534123/LConn1
  T_130534123__/RConn2 -- L_130534123/LConn2
  L_130534123/LConn3 -- T_130534123__/RConn3 -- bus314/LConn1
  T_373906159_110000_Княженская/RConn1 -- L_373906159/LConn1
  T_373906159_110000_Княженская/RConn2 -- L_373906159/LConn2
  L_373906159/LConn3 -- T_373906159_110000_Княженская/RConn3 -- bus315/LConn1
  T_144699678_110000_Новогеоргиевская/RConn1 -- L_144699678/LConn1
  T_144699678_110000_Новогеоргиевская/RConn2 -- L_144699678/LConn2
  L_144699678/LConn3 -- T_144699678_110000_Новогеоргиевская/RConn3 -- bus316/LConn1
  T_114429183__ПС_Первоуральская/RConn1 -- L_114429183/LConn1
  T_114429183__ПС_Первоуральская/RConn2 -- L_114429183/LConn2
  L_114429183/LConn3 -- T_114429183__ПС_Первоуральская/RConn3 -- bus317/LConn1
  T_166629221__/RConn1 -- L_166629221/LConn1
  T_166629221__/RConn2 -- L_166629221/LConn2
  L_166629221/LConn3 -- T_166629221__/RConn3 -- bus318/LConn1
  T_212739375__/RConn1 -- L_212739375/LConn1
  T_212739375__/RConn2 -- L_212739375/LConn2
  L_212739375/LConn3 -- T_212739375__/RConn3 -- bus319/LConn1
  T_119306741__/RConn1 -- L_119306741/LConn1
  T_119306741__/RConn2 -- L_119306741/LConn2
  L_119306741/LConn3 -- T_119306741__/RConn3 -- bus320/LConn1
  T_276394758_110000;6000_Твёрдые_сплавы/RConn1 -- L_276394758/LConn1
  T_276394758_110000;6000_Твёрдые_сплавы/RConn2 -- L_276394758/LConn2
  L_276394758/LConn3 -- T_276394758_110000;6000_Твёрдые_сплавы/RConn3 -- bus321/LConn1
  T_111353172__Заречная/RConn1 -- L_111353172/LConn1
  T_111353172__Заречная/RConn2 -- L_111353172/LConn2
  L_111353172/LConn3 -- T_111353172__Заречная/RConn3 -- bus322/LConn1
  T_332377360__/RConn1 -- L_332377360/LConn1
  T_332377360__/RConn2 -- L_332377360/LConn2
  L_332377360/LConn3 -- T_332377360__/RConn3 -- bus323/LConn1
  T_207569689_110000;35000;6000_ПС_Насосная/RConn1 -- L_207569689/LConn1
  T_207569689_110000;35000;6000_ПС_Насосная/RConn2 -- L_207569689/LConn2
  L_207569689/LConn3 -- T_207569689_110000;35000;6000_ПС_Насосная/RConn3 -- bus324/LConn1
  T_95452082_110000_Даурская/RConn1 -- L_95452082/LConn1
  T_95452082_110000_Даурская/RConn2 -- L_95452082/LConn2
  L_95452082/LConn3 -- T_95452082_110000_Даурская/RConn3 -- bus325/LConn1
  T_229397794_110000;10000_ПС_Тугулым/RConn1 -- L_229397794/LConn1
  T_229397794_110000;10000_ПС_Тугулым/RConn2 -- L_229397794/LConn2
  L_229397794/LConn3 -- T_229397794_110000;10000_ПС_Тугулым/RConn3 -- bus326/LConn1
  T_279664558_110000_ПС_Зарница/RConn1 -- L_279664558/LConn1
  T_279664558_110000_ПС_Зарница/RConn2 -- L_279664558/LConn2
  L_279664558/LConn3 -- T_279664558_110000_ПС_Зарница/RConn3 -- bus327/LConn1
  T_314008364_110000_Березинская/RConn1 -- L_314008364/LConn1
  T_314008364_110000_Березинская/RConn2 -- L_314008364/LConn2
  L_314008364/LConn3 -- T_314008364_110000_Березинская/RConn3 -- bus328/LConn1
  T_282748778__/RConn1 -- L_282748778/LConn1
  T_282748778__/RConn2 -- L_282748778/LConn2
  L_282748778/LConn3 -- T_282748778__/RConn3 -- bus329/LConn1
  T_282850239__/RConn1 -- L_282850239/LConn1
  T_282850239__/RConn2 -- L_282850239/LConn2
  L_282850239/LConn3 -- T_282850239__/RConn3 -- bus330/LConn1
  T_92045303__/RConn1 -- L_92045303/LConn1
  T_92045303__/RConn2 -- L_92045303/LConn2
  L_92045303/LConn3 -- T_92045303__/RConn3 -- bus331/LConn1
  T_255032299__/RConn1 -- L_255032299/LConn1
  T_255032299__/RConn2 -- L_255032299/LConn2
  L_255032299/LConn3 -- T_255032299__/RConn3 -- bus332/LConn1
  T_255032301__/RConn1 -- L_255032301/LConn1
  T_255032301__/RConn2 -- L_255032301/LConn2
  L_255032301/LConn3 -- T_255032301__/RConn3 -- bus333/LConn1
  T_189890976__ОРУ_110_кВ/RConn1 -- L_189890976/LConn1
  T_189890976__ОРУ_110_кВ/RConn2 -- L_189890976/LConn2
  L_189890976/LConn3 -- T_189890976__ОРУ_110_кВ/RConn3 -- bus334/LConn1
  T_279664559_110000_ПС_Кармак/RConn1 -- L_279664559/LConn1
  T_279664559_110000_ПС_Кармак/RConn2 -- L_279664559/LConn2
  L_279664559/LConn3 -- T_279664559_110000_ПС_Кармак/RConn3 -- bus335/LConn1
  T_174028758_110000;10000_ПС_Верховино/RConn1 -- L_174028758/LConn1
  T_174028758_110000;10000_ПС_Верховино/RConn2 -- L_174028758/LConn2
  L_174028758/LConn3 -- T_174028758_110000;10000_ПС_Верховино/RConn3 -- bus336/LConn1
  T_281458614_220000;110000_ПС_Краснотурьинск/RConn1 -- L_281458614/LConn1
  T_281458614_220000;110000_ПС_Краснотурьинск/RConn2 -- L_281458614/LConn2
  L_281458614/LConn3 -- T_281458614_220000;110000_ПС_Краснотурьинск/RConn3 -- bus337/LConn1
  T_281458615_110000;35000;6000_ПС_Североуральск/RConn1 -- L_281458615/LConn1
  T_281458615_110000;35000;6000_ПС_Североуральск/RConn2 -- L_281458615/LConn2
  L_281458615/LConn3 -- T_281458615_110000;35000;6000_ПС_Североуральск/RConn3 -- bus338/LConn1
  T_282779592__/RConn1 -- L_282779592/LConn1
  T_282779592__/RConn2 -- L_282779592/LConn2
  L_282779592/LConn3 -- T_282779592__/RConn3 -- bus339/LConn1
  T_337947383__/RConn1 -- L_337947383/LConn1
  T_337947383__/RConn2 -- L_337947383/LConn2
  L_337947383/LConn3 -- T_337947383__/RConn3 -- bus340/LConn1
  T_386978254_110000_Маякская/RConn1 -- L_386978254/LConn1
  T_386978254_110000_Маякская/RConn2 -- L_386978254/LConn2
  L_386978254/LConn3 -- T_386978254_110000_Маякская/RConn3 -- bus341/LConn1
  T_277716444_110000;10000_ПС_Успенка/RConn1 -- L_277716444/LConn1
  T_277716444_110000;10000_ПС_Успенка/RConn2 -- L_277716444/LConn2
  L_277716444/LConn3 -- T_277716444_110000;10000_ПС_Успенка/RConn3 -- bus342/LConn1
  T_108720649__/RConn1 -- L_108720649/LConn1
  T_108720649__/RConn2 -- L_108720649/LConn2
  L_108720649/LConn3 -- T_108720649__/RConn3 -- bus343/LConn1
  T_93464361__Переключательный_пункт_Сосьва/RConn1 -- L_93464361/LConn1
  T_93464361__Переключательный_пункт_Сосьва/RConn2 -- L_93464361/LConn2
  L_93464361/LConn3 -- T_93464361__Переключательный_пункт_Сосьва/RConn3 -- bus344/LConn1
  T_96989708__/RConn1 -- L_96989708/LConn1
  T_96989708__/RConn2 -- L_96989708/LConn2
  L_96989708/LConn3 -- T_96989708__/RConn3 -- bus345/LConn1
  T_81131204_500000;220000;110000;35000_ПС_Южная/RConn1 -- L_81131204/LConn1
  T_81131204_500000;220000;110000;35000_ПС_Южная/RConn2 -- L_81131204/LConn2
  L_81131204/LConn3 -- T_81131204_500000;220000;110000;35000_ПС_Южная/RConn3 -- bus346/LConn1
  T_275095874_220000_/RConn1 -- L_275095874/LConn1
  T_275095874_220000_/RConn2 -- L_275095874/LConn2
  L_275095874/LConn3 -- T_275095874_220000_/RConn3 -- bus347/LConn1
  T_274851651_220000;110000_ПС_Первомайская/RConn1 -- L_274851651/LConn1
  T_274851651_220000;110000_ПС_Первомайская/RConn2 -- L_274851651/LConn2
  L_274851651/LConn3 -- T_274851651_220000;110000_ПС_Первомайская/RConn3 -- bus348/LConn1
  T_107585072_220000_ПС_Салда/RConn1 -- L_107585072/LConn1
  T_107585072_220000_ПС_Салда/RConn2 -- L_107585072/LConn2
  L_107585072/LConn3 -- T_107585072_220000_ПС_Салда/RConn3 -- bus349/LConn1
  T_209726497_220000_Подстанция_«Васильев»/RConn1 -- L_209726497/LConn1
  T_209726497_220000_Подстанция_«Васильев»/RConn2 -- L_209726497/LConn2
  L_209726497/LConn3 -- T_209726497_220000_Подстанция_«Васильев»/RConn3 -- bus350/LConn1
  "T_239598452__Электроподстанция_220\\110\\35\"Кирьяновская\""/RConn1 -- L_239598452/LConn1
  "T_239598452__Электроподстанция_220\\110\\35\"Кирьяновская\""/RConn2 -- L_239598452/LConn2
  L_239598452/LConn3 -- "T_239598452__Электроподстанция_220\\110\\35\"Кирьяновская\""/RConn3 -- bus351/LConn1
  T_178844846__/RConn1 -- L_178844846/LConn1
  T_178844846__/RConn2 -- L_178844846/LConn2
  L_178844846/LConn3 -- T_178844846__/RConn3 -- bus352/LConn1
  T_96040535_220000_ПС_Вязовская/RConn1 -- L_96040535/LConn1
  T_96040535_220000_ПС_Вязовская/RConn2 -- L_96040535/LConn2
  L_96040535/LConn3 -- T_96040535_220000_ПС_Вязовская/RConn3 -- bus353/LConn1
  "T_349543035__ПС_\"Мираж\""/RConn1 -- L_349543035/LConn1
  "T_349543035__ПС_\"Мираж\""/RConn2 -- L_349543035/LConn2
  L_349543035/LConn3 -- "T_349543035__ПС_\"Мираж\""/RConn3 -- bus354/LConn1
  T_130503101_220000_Подстанция_«Советско_Соснинская»/RConn1 -- L_130503101/LConn1
  T_130503101_220000_Подстанция_«Советско_Соснинская»/RConn2 -- L_130503101/LConn2
  L_130503101/LConn3 -- T_130503101_220000_Подстанция_«Советско_Соснинская»/RConn3 -- bus355/LConn1
  T_86338059__/RConn1 -- L_86338059/LConn1
  T_86338059__/RConn2 -- L_86338059/LConn2
  L_86338059/LConn3 -- T_86338059__/RConn3 -- bus356/LConn1
  T_106808187__/RConn1 -- L_106808187/LConn1
  T_106808187__/RConn2 -- L_106808187/LConn2
  L_106808187/LConn3 -- T_106808187__/RConn3 -- bus357/LConn1
  T_219112642__ПС_90/RConn1 -- L_219112642/LConn1
  T_219112642__ПС_90/RConn2 -- L_219112642/LConn2
  L_219112642/LConn3 -- T_219112642__ПС_90/RConn3 -- bus358/LConn1
  T_150165502_220000_ПС_Рябина/RConn1 -- L_150165502/LConn1
  T_150165502_220000_ПС_Рябина/RConn2 -- L_150165502/LConn2
  L_150165502/LConn3 -- T_150165502_220000_ПС_Рябина/RConn3 -- bus359/LConn1
  T_300566433_220000;110000;10000_ПС_Белка/RConn1 -- L_300566433/LConn1
  T_300566433_220000;110000;10000_ПС_Белка/RConn2 -- L_300566433/LConn2
  L_300566433/LConn3 -- T_300566433_220000;110000;10000_ПС_Белка/RConn3 -- bus360/LConn1
  T_108718929_500000;220000;110000;10000_ПС_БАЗ/RConn1 -- L_108718929/LConn1
  T_108718929_500000;220000;110000;10000_ПС_БАЗ/RConn2 -- L_108718929/LConn2
  L_108718929/LConn3 -- T_108718929_500000;220000;110000;10000_ПС_БАЗ/RConn3 -- bus361/LConn1
  T_85603217__Сирень/RConn1 -- L_85603217/LConn1
  T_85603217__Сирень/RConn2 -- L_85603217/LConn2
  L_85603217/LConn3 -- T_85603217__Сирень/RConn3 -- bus362/LConn1
  T_173759594__Подстанция_Эмтор/RConn1 -- L_173759594/LConn1
  T_173759594__Подстанция_Эмтор/RConn2 -- L_173759594/LConn2
  L_173759594/LConn3 -- T_173759594__Подстанция_Эмтор/RConn3 -- bus363/LConn1
  T_149575176__/RConn1 -- L_149575176/LConn1
  T_149575176__/RConn2 -- L_149575176/LConn2
  L_149575176/LConn3 -- T_149575176__/RConn3 -- bus364/LConn1
  T_255065507_500000_Подстанция_«Тарко_Сале»/RConn1 -- L_255065507/LConn1
  T_255065507_500000_Подстанция_«Тарко_Сале»/RConn2 -- L_255065507/LConn2
  L_255065507/LConn3 -- T_255065507_500000_Подстанция_«Тарко_Сале»/RConn3 -- bus365/LConn1
  "T_145299338__Электроподстанция_\"Нелым\""/RConn1 -- L_145299338/LConn1
  "T_145299338__Электроподстанция_\"Нелым\""/RConn2 -- L_145299338/LConn2
  L_145299338/LConn3 -- "T_145299338__Электроподстанция_\"Нелым\""/RConn3 -- bus366/LConn1
  T_27258925_500000_ПС_Тюмень/RConn1 -- L_27258925/LConn1
  T_27258925_500000_ПС_Тюмень/RConn2 -- L_27258925/LConn2
  L_27258925/LConn3 -- T_27258925_500000_ПС_Тюмень/RConn3 -- bus367/LConn1
  T_145299339__Электроподстанция/RConn1 -- L_145299339/LConn1
  T_145299339__Электроподстанция/RConn2 -- L_145299339/LConn2
  L_145299339/LConn3 -- T_145299339__Электроподстанция/RConn3 -- bus368/LConn1
  T_100289117__/RConn1 -- L_100289117/LConn1
  T_100289117__/RConn2 -- L_100289117/LConn2
  L_100289117/LConn3 -- T_100289117__/RConn3 -- bus369/LConn1
  T_131369782_500000_Подстанция_«Трачуковская»/RConn1 -- L_131369782/LConn1
  T_131369782_500000_Подстанция_«Трачуковская»/RConn2 -- L_131369782/LConn2
  L_131369782/LConn3 -- T_131369782_500000_Подстанция_«Трачуковская»/RConn3 -- bus370/LConn1
  T_100978216_500000_Челябинская/RConn1 -- L_100978216/LConn1
  T_100978216_500000_Челябинская/RConn2 -- L_100978216/LConn2
  L_100978216/LConn3 -- T_100978216_500000_Челябинская/RConn3 -- bus371/LConn1
  "T_99190583_500000;220000;110000;fixme_\"Смеловская\"_500_кВ"/RConn1 -- L_99190583/LConn1
  "T_99190583_500000;220000;110000;fixme_\"Смеловская\"_500_кВ"/RConn2 -- L_99190583/LConn2
  L_99190583/LConn3 -- "T_99190583_500000;220000;110000;fixme_\"Смеловская\"_500_кВ"/RConn3 -- bus372/LConn1
  T_219112646__/RConn1 -- L_219112646/LConn1
  T_219112646__/RConn2 -- L_219112646/LConn2
  L_219112646/LConn3 -- T_219112646__/RConn3 -- bus373/LConn1
  T_117237579__/RConn1 -- L_117237579/LConn1
  T_117237579__/RConn2 -- L_117237579/LConn2
  L_117237579/LConn3 -- T_117237579__/RConn3 -- bus374/LConn1
  T_169556579__ПC_Приваловская_500_кВ/RConn1 -- L_169556579/LConn1
  T_169556579__ПC_Приваловская_500_кВ/RConn2 -- L_169556579/LConn2
  L_169556579/LConn3 -- T_169556579__ПC_Приваловская_500_кВ/RConn3 -- bus375/LConn1
  T_244062688_500000_Подстанция_«Ильково»/RConn1 -- L_244062688/LConn1
  T_244062688_500000_Подстанция_«Ильково»/RConn2 -- L_244062688/LConn2
  L_244062688/LConn3 -- T_244062688_500000_Подстанция_«Ильково»/RConn3 -- bus376/LConn1
  T_163913701__/RConn1 -- L_163913701/LConn1
  T_163913701__/RConn2 -- L_163913701/LConn2
  L_163913701/LConn3 -- T_163913701__/RConn3 -- bus377/LConn1
  T_113767652_500000_ПС_Кропачево/RConn1 -- L_113767652/LConn1
  T_113767652_500000_ПС_Кропачево/RConn2 -- L_113767652/LConn2
  L_113767652/LConn3 -- T_113767652_500000_ПС_Кропачево/RConn3 -- bus378/LConn1
